simulink model "iot_casestudy_1_32"  (R2023a)
settings: Solver=VariableStepAuto  StartTime=0.0  StopTime=3.0  RelTol=1e-3
undefined symbols (not defined in the file or in its folder): m, n
(part 1 of 3)
settings Model: SimulationMode=accelerator  PacingRate=0.089000  Creator=simon  LastModifiedBy=simon
settings DataIOCC: SignalLogging=off
settings OptimizationCC: AccelVerboseBuild=on

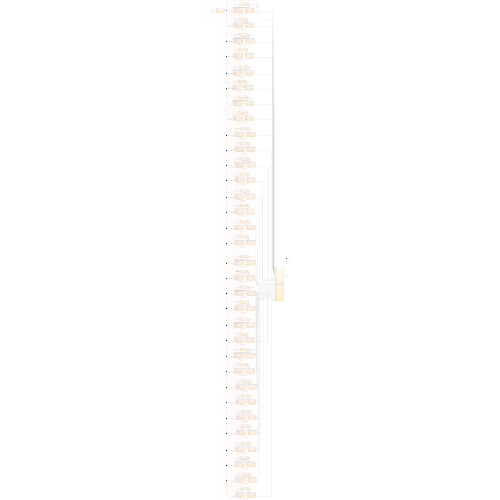
[thumbnail: Simulink's stored preview of the top-level diagram]
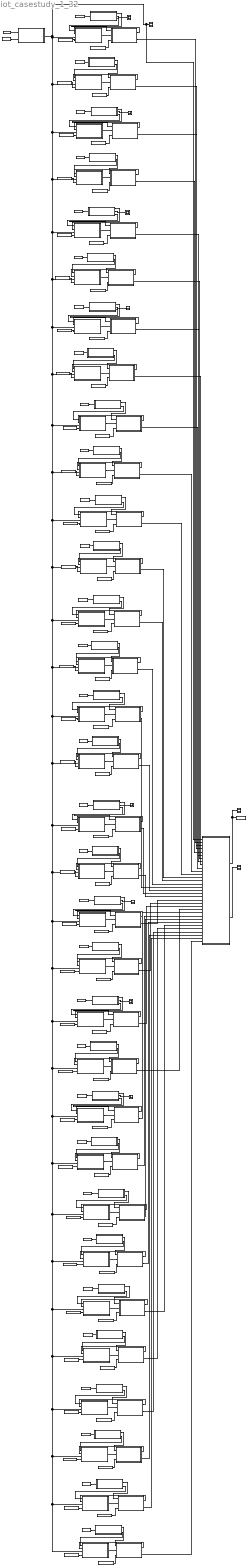
== system iot_casestudy_1_32 ==
  CameraControl : Stateflow chart  TreatAsAtomicUnit=on
      settings: PortSchema="{\"entries\":[{\"content\":{\"sides\":[{\"content\":{\"connectorIds\":[\"In3\",\"In1\",\"In2\"]},\"type\":\"ConnectorPlacement.EquallySpacedRectSide\",\"uuid\":\"ab620818-a51b-4a3c-9b00-600c4a6c30a0\"},{\"content\":{\"connectorIds\":[\"Out1\",\"Out2\"],\"side\":\"RIGHT\"},\"type\":\"ConnectorPlacement.EquallySpacedRectSide\",\"uuid\":\"fd7d4612-1aa1-44dc-acf4-0ffdcf3f06ab\"},{\"content\":{\"side\":\"TOP\"},\"type\":\"ConnectorPlacement.EquallySpacedRectSide\",\"uuid\":\"b173ad78-f658-4e97-9d6b-ed1d410de5f1\"}]},\"type\":\"ConnectorPlacement.EquallySpacedConnector\",\"uuid\":\"5700aeec-8725-4d1d-b13d-0f47828af58c\"}],\"packageUris\":[\"http://schema.mathworks.com/mf0/Connector/R2020b\"],\"version\":\"1.0\"}"
  CameraControl1 : Stateflow chart  TreatAsAtomicUnit=on
      settings: PortSchema="{\"entries\":[{\"content\":{\"sides\":[{\"content\":{\"connectorIds\":[\"In3\",\"In1\",\"In2\"]},\"type\":\"ConnectorPlacement.EquallySpacedRectSide\",\"uuid\":\"ab620818-a51b-4a3c-9b00-600c4a6c30a0\"},{\"content\":{\"connectorIds\":[\"Out1\",\"Out2\"],\"side\":\"RIGHT\"},\"type\":\"ConnectorPlacement.EquallySpacedRectSide\",\"uuid\":\"fd7d4612-1aa1-44dc-acf4-0ffdcf3f06ab\"},{\"content\":{\"side\":\"TOP\"},\"type\":\"ConnectorPlacement.EquallySpacedRectSide\",\"uuid\":\"b173ad78-f658-4e97-9d6b-ed1d410de5f1\"}]},\"type\":\"ConnectorPlacement.EquallySpacedConnector\",\"uuid\":\"5700aeec-8725-4d1d-b13d-0f47828af58c\"}],\"packageUris\":[\"http://schema.mathworks.com/mf0/Connector/R2020b\"],\"version\":\"1.0\"}"
  CameraControl10 : Stateflow chart  TreatAsAtomicUnit=on
      settings: PortSchema="{\"entries\":[{\"content\":{\"sides\":[{\"content\":{\"connectorIds\":[\"In3\",\"In1\",\"In2\"]},\"type\":\"ConnectorPlacement.EquallySpacedRectSide\",\"uuid\":\"ab620818-a51b-4a3c-9b00-600c4a6c30a0\"},{\"content\":{\"connectorIds\":[\"Out1\",\"Out2\"],\"side\":\"RIGHT\"},\"type\":\"ConnectorPlacement.EquallySpacedRectSide\",\"uuid\":\"fd7d4612-1aa1-44dc-acf4-0ffdcf3f06ab\"},{\"content\":{\"side\":\"TOP\"},\"type\":\"ConnectorPlacement.EquallySpacedRectSide\",\"uuid\":\"b173ad78-f658-4e97-9d6b-ed1d410de5f1\"}]},\"type\":\"ConnectorPlacement.EquallySpacedConnector\",\"uuid\":\"5700aeec-8725-4d1d-b13d-0f47828af58c\"}],\"packageUris\":[\"http://schema.mathworks.com/mf0/Connector/R2020b\"],\"version\":\"1.0\"}"
  CameraControl11 : Stateflow chart  TreatAsAtomicUnit=on
      settings: PortSchema="{\"entries\":[{\"content\":{\"sides\":[{\"content\":{\"connectorIds\":[\"In3\",\"In1\",\"In2\"]},\"type\":\"ConnectorPlacement.EquallySpacedRectSide\",\"uuid\":\"ab620818-a51b-4a3c-9b00-600c4a6c30a0\"},{\"content\":{\"connectorIds\":[\"Out1\",\"Out2\"],\"side\":\"RIGHT\"},\"type\":\"ConnectorPlacement.EquallySpacedRectSide\",\"uuid\":\"fd7d4612-1aa1-44dc-acf4-0ffdcf3f06ab\"},{\"content\":{\"side\":\"TOP\"},\"type\":\"ConnectorPlacement.EquallySpacedRectSide\",\"uuid\":\"b173ad78-f658-4e97-9d6b-ed1d410de5f1\"}]},\"type\":\"ConnectorPlacement.EquallySpacedConnector\",\"uuid\":\"5700aeec-8725-4d1d-b13d-0f47828af58c\"}],\"packageUris\":[\"http://schema.mathworks.com/mf0/Connector/R2020b\"],\"version\":\"1.0\"}"
  CameraControl12 : Stateflow chart  TreatAsAtomicUnit=on
      settings: PortSchema="{\"entries\":[{\"content\":{\"sides\":[{\"content\":{\"connectorIds\":[\"In3\",\"In1\",\"In2\"]},\"type\":\"ConnectorPlacement.EquallySpacedRectSide\",\"uuid\":\"ab620818-a51b-4a3c-9b00-600c4a6c30a0\"},{\"content\":{\"connectorIds\":[\"Out1\",\"Out2\"],\"side\":\"RIGHT\"},\"type\":\"ConnectorPlacement.EquallySpacedRectSide\",\"uuid\":\"fd7d4612-1aa1-44dc-acf4-0ffdcf3f06ab\"},{\"content\":{\"side\":\"TOP\"},\"type\":\"ConnectorPlacement.EquallySpacedRectSide\",\"uuid\":\"b173ad78-f658-4e97-9d6b-ed1d410de5f1\"}]},\"type\":\"ConnectorPlacement.EquallySpacedConnector\",\"uuid\":\"5700aeec-8725-4d1d-b13d-0f47828af58c\"}],\"packageUris\":[\"http://schema.mathworks.com/mf0/Connector/R2020b\"],\"version\":\"1.0\"}"
  CameraControl13 : Stateflow chart  TreatAsAtomicUnit=on
      settings: PortSchema="{\"entries\":[{\"content\":{\"sides\":[{\"content\":{\"connectorIds\":[\"In3\",\"In1\",\"In2\"]},\"type\":\"ConnectorPlacement.EquallySpacedRectSide\",\"uuid\":\"ab620818-a51b-4a3c-9b00-600c4a6c30a0\"},{\"content\":{\"connectorIds\":[\"Out1\",\"Out2\"],\"side\":\"RIGHT\"},\"type\":\"ConnectorPlacement.EquallySpacedRectSide\",\"uuid\":\"fd7d4612-1aa1-44dc-acf4-0ffdcf3f06ab\"},{\"content\":{\"side\":\"TOP\"},\"type\":\"ConnectorPlacement.EquallySpacedRectSide\",\"uuid\":\"b173ad78-f658-4e97-9d6b-ed1d410de5f1\"}]},\"type\":\"ConnectorPlacement.EquallySpacedConnector\",\"uuid\":\"5700aeec-8725-4d1d-b13d-0f47828af58c\"}],\"packageUris\":[\"http://schema.mathworks.com/mf0/Connector/R2020b\"],\"version\":\"1.0\"}"
  CameraControl14 : Stateflow chart  TreatAsAtomicUnit=on
      settings: PortSchema="{\"entries\":[{\"content\":{\"sides\":[{\"content\":{\"connectorIds\":[\"In3\",\"In1\",\"In2\"]},\"type\":\"ConnectorPlacement.EquallySpacedRectSide\",\"uuid\":\"ab620818-a51b-4a3c-9b00-600c4a6c30a0\"},{\"content\":{\"connectorIds\":[\"Out1\",\"Out2\"],\"side\":\"RIGHT\"},\"type\":\"ConnectorPlacement.EquallySpacedRectSide\",\"uuid\":\"fd7d4612-1aa1-44dc-acf4-0ffdcf3f06ab\"},{\"content\":{\"side\":\"TOP\"},\"type\":\"ConnectorPlacement.EquallySpacedRectSide\",\"uuid\":\"b173ad78-f658-4e97-9d6b-ed1d410de5f1\"}]},\"type\":\"ConnectorPlacement.EquallySpacedConnector\",\"uuid\":\"5700aeec-8725-4d1d-b13d-0f47828af58c\"}],\"packageUris\":[\"http://schema.mathworks.com/mf0/Connector/R2020b\"],\"version\":\"1.0\"}"
  CameraControl15 : Stateflow chart  TreatAsAtomicUnit=on
      settings: PortSchema="{\"entries\":[{\"content\":{\"sides\":[{\"content\":{\"connectorIds\":[\"In3\",\"In1\",\"In2\"]},\"type\":\"ConnectorPlacement.EquallySpacedRectSide\",\"uuid\":\"ab620818-a51b-4a3c-9b00-600c4a6c30a0\"},{\"content\":{\"connectorIds\":[\"Out1\",\"Out2\"],\"side\":\"RIGHT\"},\"type\":\"ConnectorPlacement.EquallySpacedRectSide\",\"uuid\":\"fd7d4612-1aa1-44dc-acf4-0ffdcf3f06ab\"},{\"content\":{\"side\":\"TOP\"},\"type\":\"ConnectorPlacement.EquallySpacedRectSide\",\"uuid\":\"b173ad78-f658-4e97-9d6b-ed1d410de5f1\"}]},\"type\":\"ConnectorPlacement.EquallySpacedConnector\",\"uuid\":\"5700aeec-8725-4d1d-b13d-0f47828af58c\"}],\"packageUris\":[\"http://schema.mathworks.com/mf0/Connector/R2020b\"],\"version\":\"1.0\"}"
  CameraControl16 : Stateflow chart  TreatAsAtomicUnit=on
      settings: PortSchema="{\"entries\":[{\"content\":{\"sides\":[{\"content\":{\"connectorIds\":[\"In3\",\"In1\",\"In2\"]},\"type\":\"ConnectorPlacement.EquallySpacedRectSide\",\"uuid\":\"ab620818-a51b-4a3c-9b00-600c4a6c30a0\"},{\"content\":{\"connectorIds\":[\"Out1\",\"Out2\"],\"side\":\"RIGHT\"},\"type\":\"ConnectorPlacement.EquallySpacedRectSide\",\"uuid\":\"fd7d4612-1aa1-44dc-acf4-0ffdcf3f06ab\"},{\"content\":{\"side\":\"TOP\"},\"type\":\"ConnectorPlacement.EquallySpacedRectSide\",\"uuid\":\"b173ad78-f658-4e97-9d6b-ed1d410de5f1\"}]},\"type\":\"ConnectorPlacement.EquallySpacedConnector\",\"uuid\":\"5700aeec-8725-4d1d-b13d-0f47828af58c\"}],\"packageUris\":[\"http://schema.mathworks.com/mf0/Connector/R2020b\"],\"version\":\"1.0\"}"
  CameraControl17 : Stateflow chart  TreatAsAtomicUnit=on
      settings: PortSchema="{\"entries\":[{\"content\":{\"sides\":[{\"content\":{\"connectorIds\":[\"In3\",\"In1\",\"In2\"]},\"type\":\"ConnectorPlacement.EquallySpacedRectSide\",\"uuid\":\"ab620818-a51b-4a3c-9b00-600c4a6c30a0\"},{\"content\":{\"connectorIds\":[\"Out1\",\"Out2\"],\"side\":\"RIGHT\"},\"type\":\"ConnectorPlacement.EquallySpacedRectSide\",\"uuid\":\"fd7d4612-1aa1-44dc-acf4-0ffdcf3f06ab\"},{\"content\":{\"side\":\"TOP\"},\"type\":\"ConnectorPlacement.EquallySpacedRectSide\",\"uuid\":\"b173ad78-f658-4e97-9d6b-ed1d410de5f1\"}]},\"type\":\"ConnectorPlacement.EquallySpacedConnector\",\"uuid\":\"5700aeec-8725-4d1d-b13d-0f47828af58c\"}],\"packageUris\":[\"http://schema.mathworks.com/mf0/Connector/R2020b\"],\"version\":\"1.0\"}"
  CameraControl18 : Stateflow chart  TreatAsAtomicUnit=on
      settings: PortSchema="{\"entries\":[{\"content\":{\"sides\":[{\"content\":{\"connectorIds\":[\"In3\",\"In1\",\"In2\"]},\"type\":\"ConnectorPlacement.EquallySpacedRectSide\",\"uuid\":\"ab620818-a51b-4a3c-9b00-600c4a6c30a0\"},{\"content\":{\"connectorIds\":[\"Out1\",\"Out2\"],\"side\":\"RIGHT\"},\"type\":\"ConnectorPlacement.EquallySpacedRectSide\",\"uuid\":\"fd7d4612-1aa1-44dc-acf4-0ffdcf3f06ab\"},{\"content\":{\"side\":\"TOP\"},\"type\":\"ConnectorPlacement.EquallySpacedRectSide\",\"uuid\":\"b173ad78-f658-4e97-9d6b-ed1d410de5f1\"}]},\"type\":\"ConnectorPlacement.EquallySpacedConnector\",\"uuid\":\"5700aeec-8725-4d1d-b13d-0f47828af58c\"}],\"packageUris\":[\"http://schema.mathworks.com/mf0/Connector/R2020b\"],\"version\":\"1.0\"}"
  CameraControl19 : Stateflow chart  TreatAsAtomicUnit=on
      settings: PortSchema="{\"entries\":[{\"content\":{\"sides\":[{\"content\":{\"connectorIds\":[\"In3\",\"In1\",\"In2\"]},\"type\":\"ConnectorPlacement.EquallySpacedRectSide\",\"uuid\":\"ab620818-a51b-4a3c-9b00-600c4a6c30a0\"},{\"content\":{\"connectorIds\":[\"Out1\",\"Out2\"],\"side\":\"RIGHT\"},\"type\":\"ConnectorPlacement.EquallySpacedRectSide\",\"uuid\":\"fd7d4612-1aa1-44dc-acf4-0ffdcf3f06ab\"},{\"content\":{\"side\":\"TOP\"},\"type\":\"ConnectorPlacement.EquallySpacedRectSide\",\"uuid\":\"b173ad78-f658-4e97-9d6b-ed1d410de5f1\"}]},\"type\":\"ConnectorPlacement.EquallySpacedConnector\",\"uuid\":\"5700aeec-8725-4d1d-b13d-0f47828af58c\"}],\"packageUris\":[\"http://schema.mathworks.com/mf0/Connector/R2020b\"],\"version\":\"1.0\"}"
  CameraControl2 : Stateflow chart  TreatAsAtomicUnit=on
      settings: PortSchema="{\"entries\":[{\"content\":{\"sides\":[{\"content\":{\"connectorIds\":[\"In3\",\"In1\",\"In2\"]},\"type\":\"ConnectorPlacement.EquallySpacedRectSide\",\"uuid\":\"ab620818-a51b-4a3c-9b00-600c4a6c30a0\"},{\"content\":{\"connectorIds\":[\"Out1\",\"Out2\"],\"side\":\"RIGHT\"},\"type\":\"ConnectorPlacement.EquallySpacedRectSide\",\"uuid\":\"fd7d4612-1aa1-44dc-acf4-0ffdcf3f06ab\"},{\"content\":{\"side\":\"TOP\"},\"type\":\"ConnectorPlacement.EquallySpacedRectSide\",\"uuid\":\"b173ad78-f658-4e97-9d6b-ed1d410de5f1\"}]},\"type\":\"ConnectorPlacement.EquallySpacedConnector\",\"uuid\":\"5700aeec-8725-4d1d-b13d-0f47828af58c\"}],\"packageUris\":[\"http://schema.mathworks.com/mf0/Connector/R2020b\"],\"version\":\"1.0\"}"
  CameraControl20 : Stateflow chart  TreatAsAtomicUnit=on
      settings: PortSchema="{\"entries\":[{\"content\":{\"sides\":[{\"content\":{\"connectorIds\":[\"In3\",\"In1\",\"In2\"]},\"type\":\"ConnectorPlacement.EquallySpacedRectSide\",\"uuid\":\"ab620818-a51b-4a3c-9b00-600c4a6c30a0\"},{\"content\":{\"connectorIds\":[\"Out1\",\"Out2\"],\"side\":\"RIGHT\"},\"type\":\"ConnectorPlacement.EquallySpacedRectSide\",\"uuid\":\"fd7d4612-1aa1-44dc-acf4-0ffdcf3f06ab\"},{\"content\":{\"side\":\"TOP\"},\"type\":\"ConnectorPlacement.EquallySpacedRectSide\",\"uuid\":\"b173ad78-f658-4e97-9d6b-ed1d410de5f1\"}]},\"type\":\"ConnectorPlacement.EquallySpacedConnector\",\"uuid\":\"5700aeec-8725-4d1d-b13d-0f47828af58c\"}],\"packageUris\":[\"http://schema.mathworks.com/mf0/Connector/R2020b\"],\"version\":\"1.0\"}"
  CameraControl21 : Stateflow chart  TreatAsAtomicUnit=on
      settings: PortSchema="{\"entries\":[{\"content\":{\"sides\":[{\"content\":{\"connectorIds\":[\"In3\",\"In1\",\"In2\"]},\"type\":\"ConnectorPlacement.EquallySpacedRectSide\",\"uuid\":\"ab620818-a51b-4a3c-9b00-600c4a6c30a0\"},{\"content\":{\"connectorIds\":[\"Out1\",\"Out2\"],\"side\":\"RIGHT\"},\"type\":\"ConnectorPlacement.EquallySpacedRectSide\",\"uuid\":\"fd7d4612-1aa1-44dc-acf4-0ffdcf3f06ab\"},{\"content\":{\"side\":\"TOP\"},\"type\":\"ConnectorPlacement.EquallySpacedRectSide\",\"uuid\":\"b173ad78-f658-4e97-9d6b-ed1d410de5f1\"}]},\"type\":\"ConnectorPlacement.EquallySpacedConnector\",\"uuid\":\"5700aeec-8725-4d1d-b13d-0f47828af58c\"}],\"packageUris\":[\"http://schema.mathworks.com/mf0/Connector/R2020b\"],\"version\":\"1.0\"}"
  CameraControl22 : Stateflow chart  TreatAsAtomicUnit=on
      settings: PortSchema="{\"entries\":[{\"content\":{\"sides\":[{\"content\":{\"connectorIds\":[\"In3\",\"In1\",\"In2\"]},\"type\":\"ConnectorPlacement.EquallySpacedRectSide\",\"uuid\":\"ab620818-a51b-4a3c-9b00-600c4a6c30a0\"},{\"content\":{\"connectorIds\":[\"Out1\",\"Out2\"],\"side\":\"RIGHT\"},\"type\":\"ConnectorPlacement.EquallySpacedRectSide\",\"uuid\":\"fd7d4612-1aa1-44dc-acf4-0ffdcf3f06ab\"},{\"content\":{\"side\":\"TOP\"},\"type\":\"ConnectorPlacement.EquallySpacedRectSide\",\"uuid\":\"b173ad78-f658-4e97-9d6b-ed1d410de5f1\"}]},\"type\":\"ConnectorPlacement.EquallySpacedConnector\",\"uuid\":\"5700aeec-8725-4d1d-b13d-0f47828af58c\"}],\"packageUris\":[\"http://schema.mathworks.com/mf0/Connector/R2020b\"],\"version\":\"1.0\"}"
  CameraControl23 : Stateflow chart  TreatAsAtomicUnit=on
      settings: PortSchema="{\"entries\":[{\"content\":{\"sides\":[{\"content\":{\"connectorIds\":[\"In3\",\"In1\",\"In2\"]},\"type\":\"ConnectorPlacement.EquallySpacedRectSide\",\"uuid\":\"ab620818-a51b-4a3c-9b00-600c4a6c30a0\"},{\"content\":{\"connectorIds\":[\"Out1\",\"Out2\"],\"side\":\"RIGHT\"},\"type\":\"ConnectorPlacement.EquallySpacedRectSide\",\"uuid\":\"fd7d4612-1aa1-44dc-acf4-0ffdcf3f06ab\"},{\"content\":{\"side\":\"TOP\"},\"type\":\"ConnectorPlacement.EquallySpacedRectSide\",\"uuid\":\"b173ad78-f658-4e97-9d6b-ed1d410de5f1\"}]},\"type\":\"ConnectorPlacement.EquallySpacedConnector\",\"uuid\":\"5700aeec-8725-4d1d-b13d-0f47828af58c\"}],\"packageUris\":[\"http://schema.mathworks.com/mf0/Connector/R2020b\"],\"version\":\"1.0\"}"
  CameraControl24 : Stateflow chart  TreatAsAtomicUnit=on
      settings: PortSchema="{\"entries\":[{\"content\":{\"sides\":[{\"content\":{\"connectorIds\":[\"In3\",\"In1\",\"In2\"]},\"type\":\"ConnectorPlacement.EquallySpacedRectSide\",\"uuid\":\"ab620818-a51b-4a3c-9b00-600c4a6c30a0\"},{\"content\":{\"connectorIds\":[\"Out1\",\"Out2\"],\"side\":\"RIGHT\"},\"type\":\"ConnectorPlacement.EquallySpacedRectSide\",\"uuid\":\"fd7d4612-1aa1-44dc-acf4-0ffdcf3f06ab\"},{\"content\":{\"side\":\"TOP\"},\"type\":\"ConnectorPlacement.EquallySpacedRectSide\",\"uuid\":\"b173ad78-f658-4e97-9d6b-ed1d410de5f1\"}]},\"type\":\"ConnectorPlacement.EquallySpacedConnector\",\"uuid\":\"5700aeec-8725-4d1d-b13d-0f47828af58c\"}],\"packageUris\":[\"http://schema.mathworks.com/mf0/Connector/R2020b\"],\"version\":\"1.0\"}"
  CameraControl25 : Stateflow chart  TreatAsAtomicUnit=on
      settings: PortSchema="{\"entries\":[{\"content\":{\"sides\":[{\"content\":{\"connectorIds\":[\"In3\",\"In1\",\"In2\"]},\"type\":\"ConnectorPlacement.EquallySpacedRectSide\",\"uuid\":\"ab620818-a51b-4a3c-9b00-600c4a6c30a0\"},{\"content\":{\"connectorIds\":[\"Out1\",\"Out2\"],\"side\":\"RIGHT\"},\"type\":\"ConnectorPlacement.EquallySpacedRectSide\",\"uuid\":\"fd7d4612-1aa1-44dc-acf4-0ffdcf3f06ab\"},{\"content\":{\"side\":\"TOP\"},\"type\":\"ConnectorPlacement.EquallySpacedRectSide\",\"uuid\":\"b173ad78-f658-4e97-9d6b-ed1d410de5f1\"}]},\"type\":\"ConnectorPlacement.EquallySpacedConnector\",\"uuid\":\"5700aeec-8725-4d1d-b13d-0f47828af58c\"}],\"packageUris\":[\"http://schema.mathworks.com/mf0/Connector/R2020b\"],\"version\":\"1.0\"}"
  CameraControl26 : Stateflow chart  TreatAsAtomicUnit=on
      settings: PortSchema="{\"entries\":[{\"content\":{\"sides\":[{\"content\":{\"connectorIds\":[\"In3\",\"In1\",\"In2\"]},\"type\":\"ConnectorPlacement.EquallySpacedRectSide\",\"uuid\":\"ab620818-a51b-4a3c-9b00-600c4a6c30a0\"},{\"content\":{\"connectorIds\":[\"Out1\",\"Out2\"],\"side\":\"RIGHT\"},\"type\":\"ConnectorPlacement.EquallySpacedRectSide\",\"uuid\":\"fd7d4612-1aa1-44dc-acf4-0ffdcf3f06ab\"},{\"content\":{\"side\":\"TOP\"},\"type\":\"ConnectorPlacement.EquallySpacedRectSide\",\"uuid\":\"b173ad78-f658-4e97-9d6b-ed1d410de5f1\"}]},\"type\":\"ConnectorPlacement.EquallySpacedConnector\",\"uuid\":\"5700aeec-8725-4d1d-b13d-0f47828af58c\"}],\"packageUris\":[\"http://schema.mathworks.com/mf0/Connector/R2020b\"],\"version\":\"1.0\"}"
  CameraControl27 : Stateflow chart  TreatAsAtomicUnit=on
      settings: PortSchema="{\"entries\":[{\"content\":{\"sides\":[{\"content\":{\"connectorIds\":[\"In3\",\"In1\",\"In2\"]},\"type\":\"ConnectorPlacement.EquallySpacedRectSide\",\"uuid\":\"ab620818-a51b-4a3c-9b00-600c4a6c30a0\"},{\"content\":{\"connectorIds\":[\"Out1\",\"Out2\"],\"side\":\"RIGHT\"},\"type\":\"ConnectorPlacement.EquallySpacedRectSide\",\"uuid\":\"fd7d4612-1aa1-44dc-acf4-0ffdcf3f06ab\"},{\"content\":{\"side\":\"TOP\"},\"type\":\"ConnectorPlacement.EquallySpacedRectSide\",\"uuid\":\"b173ad78-f658-4e97-9d6b-ed1d410de5f1\"}]},\"type\":\"ConnectorPlacement.EquallySpacedConnector\",\"uuid\":\"5700aeec-8725-4d1d-b13d-0f47828af58c\"}],\"packageUris\":[\"http://schema.mathworks.com/mf0/Connector/R2020b\"],\"version\":\"1.0\"}"
  CameraControl28 : Stateflow chart  TreatAsAtomicUnit=on
      settings: PortSchema="{\"entries\":[{\"content\":{\"sides\":[{\"content\":{\"connectorIds\":[\"In3\",\"In1\",\"In2\"]},\"type\":\"ConnectorPlacement.EquallySpacedRectSide\",\"uuid\":\"ab620818-a51b-4a3c-9b00-600c4a6c30a0\"},{\"content\":{\"connectorIds\":[\"Out1\",\"Out2\"],\"side\":\"RIGHT\"},\"type\":\"ConnectorPlacement.EquallySpacedRectSide\",\"uuid\":\"fd7d4612-1aa1-44dc-acf4-0ffdcf3f06ab\"},{\"content\":{\"side\":\"TOP\"},\"type\":\"ConnectorPlacement.EquallySpacedRectSide\",\"uuid\":\"b173ad78-f658-4e97-9d6b-ed1d410de5f1\"}]},\"type\":\"ConnectorPlacement.EquallySpacedConnector\",\"uuid\":\"5700aeec-8725-4d1d-b13d-0f47828af58c\"}],\"packageUris\":[\"http://schema.mathworks.com/mf0/Connector/R2020b\"],\"version\":\"1.0\"}"
  CameraControl29 : Stateflow chart  TreatAsAtomicUnit=on
      settings: PortSchema="{\"entries\":[{\"content\":{\"sides\":[{\"content\":{\"connectorIds\":[\"In3\",\"In1\",\"In2\"]},\"type\":\"ConnectorPlacement.EquallySpacedRectSide\",\"uuid\":\"ab620818-a51b-4a3c-9b00-600c4a6c30a0\"},{\"content\":{\"connectorIds\":[\"Out1\",\"Out2\"],\"side\":\"RIGHT\"},\"type\":\"ConnectorPlacement.EquallySpacedRectSide\",\"uuid\":\"fd7d4612-1aa1-44dc-acf4-0ffdcf3f06ab\"},{\"content\":{\"side\":\"TOP\"},\"type\":\"ConnectorPlacement.EquallySpacedRectSide\",\"uuid\":\"b173ad78-f658-4e97-9d6b-ed1d410de5f1\"}]},\"type\":\"ConnectorPlacement.EquallySpacedConnector\",\"uuid\":\"5700aeec-8725-4d1d-b13d-0f47828af58c\"}],\"packageUris\":[\"http://schema.mathworks.com/mf0/Connector/R2020b\"],\"version\":\"1.0\"}"
  CameraControl3 : Stateflow chart  TreatAsAtomicUnit=on
      settings: PortSchema="{\"entries\":[{\"content\":{\"sides\":[{\"content\":{\"connectorIds\":[\"In3\",\"In1\",\"In2\"]},\"type\":\"ConnectorPlacement.EquallySpacedRectSide\",\"uuid\":\"ab620818-a51b-4a3c-9b00-600c4a6c30a0\"},{\"content\":{\"connectorIds\":[\"Out1\",\"Out2\"],\"side\":\"RIGHT\"},\"type\":\"ConnectorPlacement.EquallySpacedRectSide\",\"uuid\":\"fd7d4612-1aa1-44dc-acf4-0ffdcf3f06ab\"},{\"content\":{\"side\":\"TOP\"},\"type\":\"ConnectorPlacement.EquallySpacedRectSide\",\"uuid\":\"b173ad78-f658-4e97-9d6b-ed1d410de5f1\"}]},\"type\":\"ConnectorPlacement.EquallySpacedConnector\",\"uuid\":\"5700aeec-8725-4d1d-b13d-0f47828af58c\"}],\"packageUris\":[\"http://schema.mathworks.com/mf0/Connector/R2020b\"],\"version\":\"1.0\"}"
  CameraControl30 : Stateflow chart  TreatAsAtomicUnit=on
      settings: PortSchema="{\"entries\":[{\"content\":{\"sides\":[{\"content\":{\"connectorIds\":[\"In3\",\"In1\",\"In2\"]},\"type\":\"ConnectorPlacement.EquallySpacedRectSide\",\"uuid\":\"ab620818-a51b-4a3c-9b00-600c4a6c30a0\"},{\"content\":{\"connectorIds\":[\"Out1\",\"Out2\"],\"side\":\"RIGHT\"},\"type\":\"ConnectorPlacement.EquallySpacedRectSide\",\"uuid\":\"fd7d4612-1aa1-44dc-acf4-0ffdcf3f06ab\"},{\"content\":{\"side\":\"TOP\"},\"type\":\"ConnectorPlacement.EquallySpacedRectSide\",\"uuid\":\"b173ad78-f658-4e97-9d6b-ed1d410de5f1\"}]},\"type\":\"ConnectorPlacement.EquallySpacedConnector\",\"uuid\":\"5700aeec-8725-4d1d-b13d-0f47828af58c\"}],\"packageUris\":[\"http://schema.mathworks.com/mf0/Connector/R2020b\"],\"version\":\"1.0\"}"
  CameraControl31 : Stateflow chart  TreatAsAtomicUnit=on
      settings: PortSchema="{\"entries\":[{\"content\":{\"sides\":[{\"content\":{\"connectorIds\":[\"In3\",\"In1\",\"In2\"]},\"type\":\"ConnectorPlacement.EquallySpacedRectSide\",\"uuid\":\"ab620818-a51b-4a3c-9b00-600c4a6c30a0\"},{\"content\":{\"connectorIds\":[\"Out1\",\"Out2\"],\"side\":\"RIGHT\"},\"type\":\"ConnectorPlacement.EquallySpacedRectSide\",\"uuid\":\"fd7d4612-1aa1-44dc-acf4-0ffdcf3f06ab\"},{\"content\":{\"side\":\"TOP\"},\"type\":\"ConnectorPlacement.EquallySpacedRectSide\",\"uuid\":\"b173ad78-f658-4e97-9d6b-ed1d410de5f1\"}]},\"type\":\"ConnectorPlacement.EquallySpacedConnector\",\"uuid\":\"5700aeec-8725-4d1d-b13d-0f47828af58c\"}],\"packageUris\":[\"http://schema.mathworks.com/mf0/Connector/R2020b\"],\"version\":\"1.0\"}"
  CameraControl4 : Stateflow chart  TreatAsAtomicUnit=on
      settings: PortSchema="{\"entries\":[{\"content\":{\"sides\":[{\"content\":{\"connectorIds\":[\"In3\",\"In1\",\"In2\"]},\"type\":\"ConnectorPlacement.EquallySpacedRectSide\",\"uuid\":\"ab620818-a51b-4a3c-9b00-600c4a6c30a0\"},{\"content\":{\"connectorIds\":[\"Out1\",\"Out2\"],\"side\":\"RIGHT\"},\"type\":\"ConnectorPlacement.EquallySpacedRectSide\",\"uuid\":\"fd7d4612-1aa1-44dc-acf4-0ffdcf3f06ab\"},{\"content\":{\"side\":\"TOP\"},\"type\":\"ConnectorPlacement.EquallySpacedRectSide\",\"uuid\":\"b173ad78-f658-4e97-9d6b-ed1d410de5f1\"}]},\"type\":\"ConnectorPlacement.EquallySpacedConnector\",\"uuid\":\"5700aeec-8725-4d1d-b13d-0f47828af58c\"}],\"packageUris\":[\"http://schema.mathworks.com/mf0/Connector/R2020b\"],\"version\":\"1.0\"}"
  CameraControl5 : Stateflow chart  TreatAsAtomicUnit=on
      settings: PortSchema="{\"entries\":[{\"content\":{\"sides\":[{\"content\":{\"connectorIds\":[\"In3\",\"In1\",\"In2\"]},\"type\":\"ConnectorPlacement.EquallySpacedRectSide\",\"uuid\":\"ab620818-a51b-4a3c-9b00-600c4a6c30a0\"},{\"content\":{\"connectorIds\":[\"Out1\",\"Out2\"],\"side\":\"RIGHT\"},\"type\":\"ConnectorPlacement.EquallySpacedRectSide\",\"uuid\":\"fd7d4612-1aa1-44dc-acf4-0ffdcf3f06ab\"},{\"content\":{\"side\":\"TOP\"},\"type\":\"ConnectorPlacement.EquallySpacedRectSide\",\"uuid\":\"b173ad78-f658-4e97-9d6b-ed1d410de5f1\"}]},\"type\":\"ConnectorPlacement.EquallySpacedConnector\",\"uuid\":\"5700aeec-8725-4d1d-b13d-0f47828af58c\"}],\"packageUris\":[\"http://schema.mathworks.com/mf0/Connector/R2020b\"],\"version\":\"1.0\"}"
  CameraControl6 : Stateflow chart  TreatAsAtomicUnit=on
      settings: PortSchema="{\"entries\":[{\"content\":{\"sides\":[{\"content\":{\"connectorIds\":[\"In3\",\"In1\",\"In2\"]},\"type\":\"ConnectorPlacement.EquallySpacedRectSide\",\"uuid\":\"ab620818-a51b-4a3c-9b00-600c4a6c30a0\"},{\"content\":{\"connectorIds\":[\"Out1\",\"Out2\"],\"side\":\"RIGHT\"},\"type\":\"ConnectorPlacement.EquallySpacedRectSide\",\"uuid\":\"fd7d4612-1aa1-44dc-acf4-0ffdcf3f06ab\"},{\"content\":{\"side\":\"TOP\"},\"type\":\"ConnectorPlacement.EquallySpacedRectSide\",\"uuid\":\"b173ad78-f658-4e97-9d6b-ed1d410de5f1\"}]},\"type\":\"ConnectorPlacement.EquallySpacedConnector\",\"uuid\":\"5700aeec-8725-4d1d-b13d-0f47828af58c\"}],\"packageUris\":[\"http://schema.mathworks.com/mf0/Connector/R2020b\"],\"version\":\"1.0\"}"
  CameraControl7 : Stateflow chart  TreatAsAtomicUnit=on
      settings: PortSchema="{\"entries\":[{\"content\":{\"sides\":[{\"content\":{\"connectorIds\":[\"In3\",\"In1\",\"In2\"]},\"type\":\"ConnectorPlacement.EquallySpacedRectSide\",\"uuid\":\"ab620818-a51b-4a3c-9b00-600c4a6c30a0\"},{\"content\":{\"connectorIds\":[\"Out1\",\"Out2\"],\"side\":\"RIGHT\"},\"type\":\"ConnectorPlacement.EquallySpacedRectSide\",\"uuid\":\"fd7d4612-1aa1-44dc-acf4-0ffdcf3f06ab\"},{\"content\":{\"side\":\"TOP\"},\"type\":\"ConnectorPlacement.EquallySpacedRectSide\",\"uuid\":\"b173ad78-f658-4e97-9d6b-ed1d410de5f1\"}]},\"type\":\"ConnectorPlacement.EquallySpacedConnector\",\"uuid\":\"5700aeec-8725-4d1d-b13d-0f47828af58c\"}],\"packageUris\":[\"http://schema.mathworks.com/mf0/Connector/R2020b\"],\"version\":\"1.0\"}"
  CameraControl8 : Stateflow chart  TreatAsAtomicUnit=on
      settings: PortSchema="{\"entries\":[{\"content\":{\"sides\":[{\"content\":{\"connectorIds\":[\"In3\",\"In1\",\"In2\"]},\"type\":\"ConnectorPlacement.EquallySpacedRectSide\",\"uuid\":\"ab620818-a51b-4a3c-9b00-600c4a6c30a0\"},{\"content\":{\"connectorIds\":[\"Out1\",\"Out2\"],\"side\":\"RIGHT\"},\"type\":\"ConnectorPlacement.EquallySpacedRectSide\",\"uuid\":\"fd7d4612-1aa1-44dc-acf4-0ffdcf3f06ab\"},{\"content\":{\"side\":\"TOP\"},\"type\":\"ConnectorPlacement.EquallySpacedRectSide\",\"uuid\":\"b173ad78-f658-4e97-9d6b-ed1d410de5f1\"}]},\"type\":\"ConnectorPlacement.EquallySpacedConnector\",\"uuid\":\"5700aeec-8725-4d1d-b13d-0f47828af58c\"}],\"packageUris\":[\"http://schema.mathworks.com/mf0/Connector/R2020b\"],\"version\":\"1.0\"}"
  CameraControl9 : Stateflow chart  TreatAsAtomicUnit=on
      settings: PortSchema="{\"entries\":[{\"content\":{\"sides\":[{\"content\":{\"connectorIds\":[\"In3\",\"In1\",\"In2\"]},\"type\":\"ConnectorPlacement.EquallySpacedRectSide\",\"uuid\":\"ab620818-a51b-4a3c-9b00-600c4a6c30a0\"},{\"content\":{\"connectorIds\":[\"Out1\",\"Out2\"],\"side\":\"RIGHT\"},\"type\":\"ConnectorPlacement.EquallySpacedRectSide\",\"uuid\":\"fd7d4612-1aa1-44dc-acf4-0ffdcf3f06ab\"},{\"content\":{\"side\":\"TOP\"},\"type\":\"ConnectorPlacement.EquallySpacedRectSide\",\"uuid\":\"b173ad78-f658-4e97-9d6b-ed1d410de5f1\"}]},\"type\":\"ConnectorPlacement.EquallySpacedConnector\",\"uuid\":\"5700aeec-8725-4d1d-b13d-0f47828af58c\"}],\"packageUris\":[\"http://schema.mathworks.com/mf0/Connector/R2020b\"],\"version\":\"1.0\"}"
  CameraDriver : Stateflow chart  TreatAsAtomicUnit=on
      settings: PortSchema="{\"entries\":[{\"content\":{\"sides\":[{\"content\":{\"connectorIds\":[\"In4\",\"In1\",\"In2\",\"In3\"]},\"type\":\"ConnectorPlacement.EquallySpacedRectSide\",\"uuid\":\"49bdffc0-8e15-4462-b991-b36534669558\"},{\"content\":{\"connectorIds\":[\"Out1\"],\"side\":\"RIGHT\"},\"type\":\"ConnectorPlacement.EquallySpacedRectSide\",\"uuid\":\"379950e5-a8e3-41fb-8f45-c3d731cfbd8a\"},{\"content\":{\"side\":\"TOP\"},\"type\":\"ConnectorPlacement.EquallySpacedRectSide\",\"uuid\":\"38309075-1b62-4fbc-9171-ddac584f70df\"}]},\"type\":\"ConnectorPlacement.EquallySpacedConnector\",\"uuid\":\"335a78c7-f6bb-4aff-a350-269f860e2554\"}],\"packageUris\":[\"http://schema.mathworks.com/mf0/Connector/R2020b\"],\"version\":\"1.0\"}"
  CameraDriver1 : Stateflow chart  TreatAsAtomicUnit=on
      settings: PortSchema="{\"entries\":[{\"content\":{\"sides\":[{\"content\":{\"connectorIds\":[\"In4\",\"In1\",\"In2\",\"In3\"]},\"type\":\"ConnectorPlacement.EquallySpacedRectSide\",\"uuid\":\"49bdffc0-8e15-4462-b991-b36534669558\"},{\"content\":{\"connectorIds\":[\"Out1\"],\"side\":\"RIGHT\"},\"type\":\"ConnectorPlacement.EquallySpacedRectSide\",\"uuid\":\"379950e5-a8e3-41fb-8f45-c3d731cfbd8a\"},{\"content\":{\"side\":\"TOP\"},\"type\":\"ConnectorPlacement.EquallySpacedRectSide\",\"uuid\":\"38309075-1b62-4fbc-9171-ddac584f70df\"}]},\"type\":\"ConnectorPlacement.EquallySpacedConnector\",\"uuid\":\"335a78c7-f6bb-4aff-a350-269f860e2554\"}],\"packageUris\":[\"http://schema.mathworks.com/mf0/Connector/R2020b\"],\"version\":\"1.0\"}"
  CameraDriver10 : Stateflow chart  TreatAsAtomicUnit=on
      settings: PortSchema="{\"entries\":[{\"content\":{\"sides\":[{\"content\":{\"connectorIds\":[\"In4\",\"In1\",\"In2\",\"In3\"]},\"type\":\"ConnectorPlacement.EquallySpacedRectSide\",\"uuid\":\"49bdffc0-8e15-4462-b991-b36534669558\"},{\"content\":{\"connectorIds\":[\"Out1\"],\"side\":\"RIGHT\"},\"type\":\"ConnectorPlacement.EquallySpacedRectSide\",\"uuid\":\"379950e5-a8e3-41fb-8f45-c3d731cfbd8a\"},{\"content\":{\"side\":\"TOP\"},\"type\":\"ConnectorPlacement.EquallySpacedRectSide\",\"uuid\":\"38309075-1b62-4fbc-9171-ddac584f70df\"}]},\"type\":\"ConnectorPlacement.EquallySpacedConnector\",\"uuid\":\"335a78c7-f6bb-4aff-a350-269f860e2554\"}],\"packageUris\":[\"http://schema.mathworks.com/mf0/Connector/R2020b\"],\"version\":\"1.0\"}"
  CameraDriver11 : Stateflow chart  TreatAsAtomicUnit=on
      settings: PortSchema="{\"entries\":[{\"content\":{\"sides\":[{\"content\":{\"connectorIds\":[\"In4\",\"In1\",\"In2\",\"In3\"]},\"type\":\"ConnectorPlacement.EquallySpacedRectSide\",\"uuid\":\"49bdffc0-8e15-4462-b991-b36534669558\"},{\"content\":{\"connectorIds\":[\"Out1\"],\"side\":\"RIGHT\"},\"type\":\"ConnectorPlacement.EquallySpacedRectSide\",\"uuid\":\"379950e5-a8e3-41fb-8f45-c3d731cfbd8a\"},{\"content\":{\"side\":\"TOP\"},\"type\":\"ConnectorPlacement.EquallySpacedRectSide\",\"uuid\":\"38309075-1b62-4fbc-9171-ddac584f70df\"}]},\"type\":\"ConnectorPlacement.EquallySpacedConnector\",\"uuid\":\"335a78c7-f6bb-4aff-a350-269f860e2554\"}],\"packageUris\":[\"http://schema.mathworks.com/mf0/Connector/R2020b\"],\"version\":\"1.0\"}"
  CameraDriver12 : Stateflow chart  TreatAsAtomicUnit=on
      settings: PortSchema="{\"entries\":[{\"content\":{\"sides\":[{\"content\":{\"connectorIds\":[\"In4\",\"In1\",\"In2\",\"In3\"]},\"type\":\"ConnectorPlacement.EquallySpacedRectSide\",\"uuid\":\"49bdffc0-8e15-4462-b991-b36534669558\"},{\"content\":{\"connectorIds\":[\"Out1\"],\"side\":\"RIGHT\"},\"type\":\"ConnectorPlacement.EquallySpacedRectSide\",\"uuid\":\"379950e5-a8e3-41fb-8f45-c3d731cfbd8a\"},{\"content\":{\"side\":\"TOP\"},\"type\":\"ConnectorPlacement.EquallySpacedRectSide\",\"uuid\":\"38309075-1b62-4fbc-9171-ddac584f70df\"}]},\"type\":\"ConnectorPlacement.EquallySpacedConnector\",\"uuid\":\"335a78c7-f6bb-4aff-a350-269f860e2554\"}],\"packageUris\":[\"http://schema.mathworks.com/mf0/Connector/R2020b\"],\"version\":\"1.0\"}"
  CameraDriver13 : Stateflow chart  TreatAsAtomicUnit=on
      settings: PortSchema="{\"entries\":[{\"content\":{\"sides\":[{\"content\":{\"connectorIds\":[\"In4\",\"In1\",\"In2\",\"In3\"]},\"type\":\"ConnectorPlacement.EquallySpacedRectSide\",\"uuid\":\"49bdffc0-8e15-4462-b991-b36534669558\"},{\"content\":{\"connectorIds\":[\"Out1\"],\"side\":\"RIGHT\"},\"type\":\"ConnectorPlacement.EquallySpacedRectSide\",\"uuid\":\"379950e5-a8e3-41fb-8f45-c3d731cfbd8a\"},{\"content\":{\"side\":\"TOP\"},\"type\":\"ConnectorPlacement.EquallySpacedRectSide\",\"uuid\":\"38309075-1b62-4fbc-9171-ddac584f70df\"}]},\"type\":\"ConnectorPlacement.EquallySpacedConnector\",\"uuid\":\"335a78c7-f6bb-4aff-a350-269f860e2554\"}],\"packageUris\":[\"http://schema.mathworks.com/mf0/Connector/R2020b\"],\"version\":\"1.0\"}"
  CameraDriver14 : Stateflow chart  TreatAsAtomicUnit=on
      settings: PortSchema="{\"entries\":[{\"content\":{\"sides\":[{\"content\":{\"connectorIds\":[\"In4\",\"In1\",\"In2\",\"In3\"]},\"type\":\"ConnectorPlacement.EquallySpacedRectSide\",\"uuid\":\"49bdffc0-8e15-4462-b991-b36534669558\"},{\"content\":{\"connectorIds\":[\"Out1\"],\"side\":\"RIGHT\"},\"type\":\"ConnectorPlacement.EquallySpacedRectSide\",\"uuid\":\"379950e5-a8e3-41fb-8f45-c3d731cfbd8a\"},{\"content\":{\"side\":\"TOP\"},\"type\":\"ConnectorPlacement.EquallySpacedRectSide\",\"uuid\":\"38309075-1b62-4fbc-9171-ddac584f70df\"}]},\"type\":\"ConnectorPlacement.EquallySpacedConnector\",\"uuid\":\"335a78c7-f6bb-4aff-a350-269f860e2554\"}],\"packageUris\":[\"http://schema.mathworks.com/mf0/Connector/R2020b\"],\"version\":\"1.0\"}"
  CameraDriver15 : Stateflow chart  TreatAsAtomicUnit=on
      settings: PortSchema="{\"entries\":[{\"content\":{\"sides\":[{\"content\":{\"connectorIds\":[\"In4\",\"In1\",\"In2\",\"In3\"]},\"type\":\"ConnectorPlacement.EquallySpacedRectSide\",\"uuid\":\"49bdffc0-8e15-4462-b991-b36534669558\"},{\"content\":{\"connectorIds\":[\"Out1\"],\"side\":\"RIGHT\"},\"type\":\"ConnectorPlacement.EquallySpacedRectSide\",\"uuid\":\"379950e5-a8e3-41fb-8f45-c3d731cfbd8a\"},{\"content\":{\"side\":\"TOP\"},\"type\":\"ConnectorPlacement.EquallySpacedRectSide\",\"uuid\":\"38309075-1b62-4fbc-9171-ddac584f70df\"}]},\"type\":\"ConnectorPlacement.EquallySpacedConnector\",\"uuid\":\"335a78c7-f6bb-4aff-a350-269f860e2554\"}],\"packageUris\":[\"http://schema.mathworks.com/mf0/Connector/R2020b\"],\"version\":\"1.0\"}"
  CameraDriver16 : Stateflow chart  TreatAsAtomicUnit=on
      settings: PortSchema="{\"entries\":[{\"content\":{\"sides\":[{\"content\":{\"connectorIds\":[\"In4\",\"In1\",\"In2\",\"In3\"]},\"type\":\"ConnectorPlacement.EquallySpacedRectSide\",\"uuid\":\"49bdffc0-8e15-4462-b991-b36534669558\"},{\"content\":{\"connectorIds\":[\"Out1\"],\"side\":\"RIGHT\"},\"type\":\"ConnectorPlacement.EquallySpacedRectSide\",\"uuid\":\"379950e5-a8e3-41fb-8f45-c3d731cfbd8a\"},{\"content\":{\"side\":\"TOP\"},\"type\":\"ConnectorPlacement.EquallySpacedRectSide\",\"uuid\":\"38309075-1b62-4fbc-9171-ddac584f70df\"}]},\"type\":\"ConnectorPlacement.EquallySpacedConnector\",\"uuid\":\"335a78c7-f6bb-4aff-a350-269f860e2554\"}],\"packageUris\":[\"http://schema.mathworks.com/mf0/Connector/R2020b\"],\"version\":\"1.0\"}"
  CameraDriver17 : Stateflow chart  TreatAsAtomicUnit=on
      settings: PortSchema="{\"entries\":[{\"content\":{\"sides\":[{\"content\":{\"connectorIds\":[\"In4\",\"In1\",\"In2\",\"In3\"]},\"type\":\"ConnectorPlacement.EquallySpacedRectSide\",\"uuid\":\"49bdffc0-8e15-4462-b991-b36534669558\"},{\"content\":{\"connectorIds\":[\"Out1\"],\"side\":\"RIGHT\"},\"type\":\"ConnectorPlacement.EquallySpacedRectSide\",\"uuid\":\"379950e5-a8e3-41fb-8f45-c3d731cfbd8a\"},{\"content\":{\"side\":\"TOP\"},\"type\":\"ConnectorPlacement.EquallySpacedRectSide\",\"uuid\":\"38309075-1b62-4fbc-9171-ddac584f70df\"}]},\"type\":\"ConnectorPlacement.EquallySpacedConnector\",\"uuid\":\"335a78c7-f6bb-4aff-a350-269f860e2554\"}],\"packageUris\":[\"http://schema.mathworks.com/mf0/Connector/R2020b\"],\"version\":\"1.0\"}"
  CameraDriver18 : Stateflow chart  TreatAsAtomicUnit=on
      settings: PortSchema="{\"entries\":[{\"content\":{\"sides\":[{\"content\":{\"connectorIds\":[\"In4\",\"In1\",\"In2\",\"In3\"]},\"type\":\"ConnectorPlacement.EquallySpacedRectSide\",\"uuid\":\"49bdffc0-8e15-4462-b991-b36534669558\"},{\"content\":{\"connectorIds\":[\"Out1\"],\"side\":\"RIGHT\"},\"type\":\"ConnectorPlacement.EquallySpacedRectSide\",\"uuid\":\"379950e5-a8e3-41fb-8f45-c3d731cfbd8a\"},{\"content\":{\"side\":\"TOP\"},\"type\":\"ConnectorPlacement.EquallySpacedRectSide\",\"uuid\":\"38309075-1b62-4fbc-9171-ddac584f70df\"}]},\"type\":\"ConnectorPlacement.EquallySpacedConnector\",\"uuid\":\"335a78c7-f6bb-4aff-a350-269f860e2554\"}],\"packageUris\":[\"http://schema.mathworks.com/mf0/Connector/R2020b\"],\"version\":\"1.0\"}"
  CameraDriver19 : Stateflow chart  TreatAsAtomicUnit=on
      settings: PortSchema="{\"entries\":[{\"content\":{\"sides\":[{\"content\":{\"connectorIds\":[\"In4\",\"In1\",\"In2\",\"In3\"]},\"type\":\"ConnectorPlacement.EquallySpacedRectSide\",\"uuid\":\"49bdffc0-8e15-4462-b991-b36534669558\"},{\"content\":{\"connectorIds\":[\"Out1\"],\"side\":\"RIGHT\"},\"type\":\"ConnectorPlacement.EquallySpacedRectSide\",\"uuid\":\"379950e5-a8e3-41fb-8f45-c3d731cfbd8a\"},{\"content\":{\"side\":\"TOP\"},\"type\":\"ConnectorPlacement.EquallySpacedRectSide\",\"uuid\":\"38309075-1b62-4fbc-9171-ddac584f70df\"}]},\"type\":\"ConnectorPlacement.EquallySpacedConnector\",\"uuid\":\"335a78c7-f6bb-4aff-a350-269f860e2554\"}],\"packageUris\":[\"http://schema.mathworks.com/mf0/Connector/R2020b\"],\"version\":\"1.0\"}"
  CameraDriver2 : Stateflow chart  TreatAsAtomicUnit=on
      settings: PortSchema="{\"entries\":[{\"content\":{\"sides\":[{\"content\":{\"connectorIds\":[\"In4\",\"In1\",\"In2\",\"In3\"]},\"type\":\"ConnectorPlacement.EquallySpacedRectSide\",\"uuid\":\"49bdffc0-8e15-4462-b991-b36534669558\"},{\"content\":{\"connectorIds\":[\"Out1\"],\"side\":\"RIGHT\"},\"type\":\"ConnectorPlacement.EquallySpacedRectSide\",\"uuid\":\"379950e5-a8e3-41fb-8f45-c3d731cfbd8a\"},{\"content\":{\"side\":\"TOP\"},\"type\":\"ConnectorPlacement.EquallySpacedRectSide\",\"uuid\":\"38309075-1b62-4fbc-9171-ddac584f70df\"}]},\"type\":\"ConnectorPlacement.EquallySpacedConnector\",\"uuid\":\"335a78c7-f6bb-4aff-a350-269f860e2554\"}],\"packageUris\":[\"http://schema.mathworks.com/mf0/Connector/R2020b\"],\"version\":\"1.0\"}"
  CameraDriver20 : Stateflow chart  TreatAsAtomicUnit=on
      settings: PortSchema="{\"entries\":[{\"content\":{\"sides\":[{\"content\":{\"connectorIds\":[\"In4\",\"In1\",\"In2\",\"In3\"]},\"type\":\"ConnectorPlacement.EquallySpacedRectSide\",\"uuid\":\"49bdffc0-8e15-4462-b991-b36534669558\"},{\"content\":{\"connectorIds\":[\"Out1\"],\"side\":\"RIGHT\"},\"type\":\"ConnectorPlacement.EquallySpacedRectSide\",\"uuid\":\"379950e5-a8e3-41fb-8f45-c3d731cfbd8a\"},{\"content\":{\"side\":\"TOP\"},\"type\":\"ConnectorPlacement.EquallySpacedRectSide\",\"uuid\":\"38309075-1b62-4fbc-9171-ddac584f70df\"}]},\"type\":\"ConnectorPlacement.EquallySpacedConnector\",\"uuid\":\"335a78c7-f6bb-4aff-a350-269f860e2554\"}],\"packageUris\":[\"http://schema.mathworks.com/mf0/Connector/R2020b\"],\"version\":\"1.0\"}"
  CameraDriver21 : Stateflow chart  TreatAsAtomicUnit=on
      settings: PortSchema="{\"entries\":[{\"content\":{\"sides\":[{\"content\":{\"connectorIds\":[\"In4\",\"In1\",\"In2\",\"In3\"]},\"type\":\"ConnectorPlacement.EquallySpacedRectSide\",\"uuid\":\"49bdffc0-8e15-4462-b991-b36534669558\"},{\"content\":{\"connectorIds\":[\"Out1\"],\"side\":\"RIGHT\"},\"type\":\"ConnectorPlacement.EquallySpacedRectSide\",\"uuid\":\"379950e5-a8e3-41fb-8f45-c3d731cfbd8a\"},{\"content\":{\"side\":\"TOP\"},\"type\":\"ConnectorPlacement.EquallySpacedRectSide\",\"uuid\":\"38309075-1b62-4fbc-9171-ddac584f70df\"}]},\"type\":\"ConnectorPlacement.EquallySpacedConnector\",\"uuid\":\"335a78c7-f6bb-4aff-a350-269f860e2554\"}],\"packageUris\":[\"http://schema.mathworks.com/mf0/Connector/R2020b\"],\"version\":\"1.0\"}"
  CameraDriver22 : Stateflow chart  TreatAsAtomicUnit=on
      settings: PortSchema="{\"entries\":[{\"content\":{\"sides\":[{\"content\":{\"connectorIds\":[\"In4\",\"In1\",\"In2\",\"In3\"]},\"type\":\"ConnectorPlacement.EquallySpacedRectSide\",\"uuid\":\"49bdffc0-8e15-4462-b991-b36534669558\"},{\"content\":{\"connectorIds\":[\"Out1\"],\"side\":\"RIGHT\"},\"type\":\"ConnectorPlacement.EquallySpacedRectSide\",\"uuid\":\"379950e5-a8e3-41fb-8f45-c3d731cfbd8a\"},{\"content\":{\"side\":\"TOP\"},\"type\":\"ConnectorPlacement.EquallySpacedRectSide\",\"uuid\":\"38309075-1b62-4fbc-9171-ddac584f70df\"}]},\"type\":\"ConnectorPlacement.EquallySpacedConnector\",\"uuid\":\"335a78c7-f6bb-4aff-a350-269f860e2554\"}],\"packageUris\":[\"http://schema.mathworks.com/mf0/Connector/R2020b\"],\"version\":\"1.0\"}"
  CameraDriver23 : Stateflow chart  TreatAsAtomicUnit=on
      settings: PortSchema="{\"entries\":[{\"content\":{\"sides\":[{\"content\":{\"connectorIds\":[\"In4\",\"In1\",\"In2\",\"In3\"]},\"type\":\"ConnectorPlacement.EquallySpacedRectSide\",\"uuid\":\"49bdffc0-8e15-4462-b991-b36534669558\"},{\"content\":{\"connectorIds\":[\"Out1\"],\"side\":\"RIGHT\"},\"type\":\"ConnectorPlacement.EquallySpacedRectSide\",\"uuid\":\"379950e5-a8e3-41fb-8f45-c3d731cfbd8a\"},{\"content\":{\"side\":\"TOP\"},\"type\":\"ConnectorPlacement.EquallySpacedRectSide\",\"uuid\":\"38309075-1b62-4fbc-9171-ddac584f70df\"}]},\"type\":\"ConnectorPlacement.EquallySpacedConnector\",\"uuid\":\"335a78c7-f6bb-4aff-a350-269f860e2554\"}],\"packageUris\":[\"http://schema.mathworks.com/mf0/Connector/R2020b\"],\"version\":\"1.0\"}"
  CameraDriver24 : Stateflow chart  TreatAsAtomicUnit=on
      settings: PortSchema="{\"entries\":[{\"content\":{\"sides\":[{\"content\":{\"connectorIds\":[\"In4\",\"In1\",\"In2\",\"In3\"]},\"type\":\"ConnectorPlacement.EquallySpacedRectSide\",\"uuid\":\"49bdffc0-8e15-4462-b991-b36534669558\"},{\"content\":{\"connectorIds\":[\"Out1\"],\"side\":\"RIGHT\"},\"type\":\"ConnectorPlacement.EquallySpacedRectSide\",\"uuid\":\"379950e5-a8e3-41fb-8f45-c3d731cfbd8a\"},{\"content\":{\"side\":\"TOP\"},\"type\":\"ConnectorPlacement.EquallySpacedRectSide\",\"uuid\":\"38309075-1b62-4fbc-9171-ddac584f70df\"}]},\"type\":\"ConnectorPlacement.EquallySpacedConnector\",\"uuid\":\"335a78c7-f6bb-4aff-a350-269f860e2554\"}],\"packageUris\":[\"http://schema.mathworks.com/mf0/Connector/R2020b\"],\"version\":\"1.0\"}"
  CameraDriver25 : Stateflow chart  TreatAsAtomicUnit=on
      settings: PortSchema="{\"entries\":[{\"content\":{\"sides\":[{\"content\":{\"connectorIds\":[\"In4\",\"In1\",\"In2\",\"In3\"]},\"type\":\"ConnectorPlacement.EquallySpacedRectSide\",\"uuid\":\"49bdffc0-8e15-4462-b991-b36534669558\"},{\"content\":{\"connectorIds\":[\"Out1\"],\"side\":\"RIGHT\"},\"type\":\"ConnectorPlacement.EquallySpacedRectSide\",\"uuid\":\"379950e5-a8e3-41fb-8f45-c3d731cfbd8a\"},{\"content\":{\"side\":\"TOP\"},\"type\":\"ConnectorPlacement.EquallySpacedRectSide\",\"uuid\":\"38309075-1b62-4fbc-9171-ddac584f70df\"}]},\"type\":\"ConnectorPlacement.EquallySpacedConnector\",\"uuid\":\"335a78c7-f6bb-4aff-a350-269f860e2554\"}],\"packageUris\":[\"http://schema.mathworks.com/mf0/Connector/R2020b\"],\"version\":\"1.0\"}"
  CameraDriver26 : Stateflow chart  TreatAsAtomicUnit=on
      settings: PortSchema="{\"entries\":[{\"content\":{\"sides\":[{\"content\":{\"connectorIds\":[\"In4\",\"In1\",\"In2\",\"In3\"]},\"type\":\"ConnectorPlacement.EquallySpacedRectSide\",\"uuid\":\"49bdffc0-8e15-4462-b991-b36534669558\"},{\"content\":{\"connectorIds\":[\"Out1\"],\"side\":\"RIGHT\"},\"type\":\"ConnectorPlacement.EquallySpacedRectSide\",\"uuid\":\"379950e5-a8e3-41fb-8f45-c3d731cfbd8a\"},{\"content\":{\"side\":\"TOP\"},\"type\":\"ConnectorPlacement.EquallySpacedRectSide\",\"uuid\":\"38309075-1b62-4fbc-9171-ddac584f70df\"}]},\"type\":\"ConnectorPlacement.EquallySpacedConnector\",\"uuid\":\"335a78c7-f6bb-4aff-a350-269f860e2554\"}],\"packageUris\":[\"http://schema.mathworks.com/mf0/Connector/R2020b\"],\"version\":\"1.0\"}"
  CameraDriver27 : Stateflow chart  TreatAsAtomicUnit=on
      settings: PortSchema="{\"entries\":[{\"content\":{\"sides\":[{\"content\":{\"connectorIds\":[\"In4\",\"In1\",\"In2\",\"In3\"]},\"type\":\"ConnectorPlacement.EquallySpacedRectSide\",\"uuid\":\"49bdffc0-8e15-4462-b991-b36534669558\"},{\"content\":{\"connectorIds\":[\"Out1\"],\"side\":\"RIGHT\"},\"type\":\"ConnectorPlacement.EquallySpacedRectSide\",\"uuid\":\"379950e5-a8e3-41fb-8f45-c3d731cfbd8a\"},{\"content\":{\"side\":\"TOP\"},\"type\":\"ConnectorPlacement.EquallySpacedRectSide\",\"uuid\":\"38309075-1b62-4fbc-9171-ddac584f70df\"}]},\"type\":\"ConnectorPlacement.EquallySpacedConnector\",\"uuid\":\"335a78c7-f6bb-4aff-a350-269f860e2554\"}],\"packageUris\":[\"http://schema.mathworks.com/mf0/Connector/R2020b\"],\"version\":\"1.0\"}"
  CameraDriver28 : Stateflow chart  TreatAsAtomicUnit=on
      settings: PortSchema="{\"entries\":[{\"content\":{\"sides\":[{\"content\":{\"connectorIds\":[\"In4\",\"In1\",\"In2\",\"In3\"]},\"type\":\"ConnectorPlacement.EquallySpacedRectSide\",\"uuid\":\"49bdffc0-8e15-4462-b991-b36534669558\"},{\"content\":{\"connectorIds\":[\"Out1\"],\"side\":\"RIGHT\"},\"type\":\"ConnectorPlacement.EquallySpacedRectSide\",\"uuid\":\"379950e5-a8e3-41fb-8f45-c3d731cfbd8a\"},{\"content\":{\"side\":\"TOP\"},\"type\":\"ConnectorPlacement.EquallySpacedRectSide\",\"uuid\":\"38309075-1b62-4fbc-9171-ddac584f70df\"}]},\"type\":\"ConnectorPlacement.EquallySpacedConnector\",\"uuid\":\"335a78c7-f6bb-4aff-a350-269f860e2554\"}],\"packageUris\":[\"http://schema.mathworks.com/mf0/Connector/R2020b\"],\"version\":\"1.0\"}"
  CameraDriver29 : Stateflow chart  TreatAsAtomicUnit=on
      settings: PortSchema="{\"entries\":[{\"content\":{\"sides\":[{\"content\":{\"connectorIds\":[\"In4\",\"In1\",\"In2\",\"In3\"]},\"type\":\"ConnectorPlacement.EquallySpacedRectSide\",\"uuid\":\"49bdffc0-8e15-4462-b991-b36534669558\"},{\"content\":{\"connectorIds\":[\"Out1\"],\"side\":\"RIGHT\"},\"type\":\"ConnectorPlacement.EquallySpacedRectSide\",\"uuid\":\"379950e5-a8e3-41fb-8f45-c3d731cfbd8a\"},{\"content\":{\"side\":\"TOP\"},\"type\":\"ConnectorPlacement.EquallySpacedRectSide\",\"uuid\":\"38309075-1b62-4fbc-9171-ddac584f70df\"}]},\"type\":\"ConnectorPlacement.EquallySpacedConnector\",\"uuid\":\"335a78c7-f6bb-4aff-a350-269f860e2554\"}],\"packageUris\":[\"http://schema.mathworks.com/mf0/Connector/R2020b\"],\"version\":\"1.0\"}"
  CameraDriver3 : Stateflow chart  TreatAsAtomicUnit=on
      settings: PortSchema="{\"entries\":[{\"content\":{\"sides\":[{\"content\":{\"connectorIds\":[\"In4\",\"In1\",\"In2\",\"In3\"]},\"type\":\"ConnectorPlacement.EquallySpacedRectSide\",\"uuid\":\"49bdffc0-8e15-4462-b991-b36534669558\"},{\"content\":{\"connectorIds\":[\"Out1\"],\"side\":\"RIGHT\"},\"type\":\"ConnectorPlacement.EquallySpacedRectSide\",\"uuid\":\"379950e5-a8e3-41fb-8f45-c3d731cfbd8a\"},{\"content\":{\"side\":\"TOP\"},\"type\":\"ConnectorPlacement.EquallySpacedRectSide\",\"uuid\":\"38309075-1b62-4fbc-9171-ddac584f70df\"}]},\"type\":\"ConnectorPlacement.EquallySpacedConnector\",\"uuid\":\"335a78c7-f6bb-4aff-a350-269f860e2554\"}],\"packageUris\":[\"http://schema.mathworks.com/mf0/Connector/R2020b\"],\"version\":\"1.0\"}"
  CameraDriver30 : Stateflow chart  TreatAsAtomicUnit=on
      settings: PortSchema="{\"entries\":[{\"content\":{\"sides\":[{\"content\":{\"connectorIds\":[\"In4\",\"In1\",\"In2\",\"In3\"]},\"type\":\"ConnectorPlacement.EquallySpacedRectSide\",\"uuid\":\"49bdffc0-8e15-4462-b991-b36534669558\"},{\"content\":{\"connectorIds\":[\"Out1\"],\"side\":\"RIGHT\"},\"type\":\"ConnectorPlacement.EquallySpacedRectSide\",\"uuid\":\"379950e5-a8e3-41fb-8f45-c3d731cfbd8a\"},{\"content\":{\"side\":\"TOP\"},\"type\":\"ConnectorPlacement.EquallySpacedRectSide\",\"uuid\":\"38309075-1b62-4fbc-9171-ddac584f70df\"}]},\"type\":\"ConnectorPlacement.EquallySpacedConnector\",\"uuid\":\"335a78c7-f6bb-4aff-a350-269f860e2554\"}],\"packageUris\":[\"http://schema.mathworks.com/mf0/Connector/R2020b\"],\"version\":\"1.0\"}"
  CameraDriver31 : Stateflow chart  TreatAsAtomicUnit=on
      settings: PortSchema="{\"entries\":[{\"content\":{\"sides\":[{\"content\":{\"connectorIds\":[\"In4\",\"In1\",\"In2\",\"In3\"]},\"type\":\"ConnectorPlacement.EquallySpacedRectSide\",\"uuid\":\"49bdffc0-8e15-4462-b991-b36534669558\"},{\"content\":{\"connectorIds\":[\"Out1\"],\"side\":\"RIGHT\"},\"type\":\"ConnectorPlacement.EquallySpacedRectSide\",\"uuid\":\"379950e5-a8e3-41fb-8f45-c3d731cfbd8a\"},{\"content\":{\"side\":\"TOP\"},\"type\":\"ConnectorPlacement.EquallySpacedRectSide\",\"uuid\":\"38309075-1b62-4fbc-9171-ddac584f70df\"}]},\"type\":\"ConnectorPlacement.EquallySpacedConnector\",\"uuid\":\"335a78c7-f6bb-4aff-a350-269f860e2554\"}],\"packageUris\":[\"http://schema.mathworks.com/mf0/Connector/R2020b\"],\"version\":\"1.0\"}"
  CameraDriver4 : Stateflow chart  TreatAsAtomicUnit=on
      settings: PortSchema="{\"entries\":[{\"content\":{\"sides\":[{\"content\":{\"connectorIds\":[\"In4\",\"In1\",\"In2\",\"In3\"]},\"type\":\"ConnectorPlacement.EquallySpacedRectSide\",\"uuid\":\"49bdffc0-8e15-4462-b991-b36534669558\"},{\"content\":{\"connectorIds\":[\"Out1\"],\"side\":\"RIGHT\"},\"type\":\"ConnectorPlacement.EquallySpacedRectSide\",\"uuid\":\"379950e5-a8e3-41fb-8f45-c3d731cfbd8a\"},{\"content\":{\"side\":\"TOP\"},\"type\":\"ConnectorPlacement.EquallySpacedRectSide\",\"uuid\":\"38309075-1b62-4fbc-9171-ddac584f70df\"}]},\"type\":\"ConnectorPlacement.EquallySpacedConnector\",\"uuid\":\"335a78c7-f6bb-4aff-a350-269f860e2554\"}],\"packageUris\":[\"http://schema.mathworks.com/mf0/Connector/R2020b\"],\"version\":\"1.0\"}"
  CameraDriver5 : Stateflow chart  TreatAsAtomicUnit=on
      settings: PortSchema="{\"entries\":[{\"content\":{\"sides\":[{\"content\":{\"connectorIds\":[\"In4\",\"In1\",\"In2\",\"In3\"]},\"type\":\"ConnectorPlacement.EquallySpacedRectSide\",\"uuid\":\"49bdffc0-8e15-4462-b991-b36534669558\"},{\"content\":{\"connectorIds\":[\"Out1\"],\"side\":\"RIGHT\"},\"type\":\"ConnectorPlacement.EquallySpacedRectSide\",\"uuid\":\"379950e5-a8e3-41fb-8f45-c3d731cfbd8a\"},{\"content\":{\"side\":\"TOP\"},\"type\":\"ConnectorPlacement.EquallySpacedRectSide\",\"uuid\":\"38309075-1b62-4fbc-9171-ddac584f70df\"}]},\"type\":\"ConnectorPlacement.EquallySpacedConnector\",\"uuid\":\"335a78c7-f6bb-4aff-a350-269f860e2554\"}],\"packageUris\":[\"http://schema.mathworks.com/mf0/Connector/R2020b\"],\"version\":\"1.0\"}"
  CameraDriver6 : Stateflow chart  TreatAsAtomicUnit=on
      settings: PortSchema="{\"entries\":[{\"content\":{\"sides\":[{\"content\":{\"connectorIds\":[\"In4\",\"In1\",\"In2\",\"In3\"]},\"type\":\"ConnectorPlacement.EquallySpacedRectSide\",\"uuid\":\"49bdffc0-8e15-4462-b991-b36534669558\"},{\"content\":{\"connectorIds\":[\"Out1\"],\"side\":\"RIGHT\"},\"type\":\"ConnectorPlacement.EquallySpacedRectSide\",\"uuid\":\"379950e5-a8e3-41fb-8f45-c3d731cfbd8a\"},{\"content\":{\"side\":\"TOP\"},\"type\":\"ConnectorPlacement.EquallySpacedRectSide\",\"uuid\":\"38309075-1b62-4fbc-9171-ddac584f70df\"}]},\"type\":\"ConnectorPlacement.EquallySpacedConnector\",\"uuid\":\"335a78c7-f6bb-4aff-a350-269f860e2554\"}],\"packageUris\":[\"http://schema.mathworks.com/mf0/Connector/R2020b\"],\"version\":\"1.0\"}"
  CameraDriver7 : Stateflow chart  TreatAsAtomicUnit=on
      settings: PortSchema="{\"entries\":[{\"content\":{\"sides\":[{\"content\":{\"connectorIds\":[\"In4\",\"In1\",\"In2\",\"In3\"]},\"type\":\"ConnectorPlacement.EquallySpacedRectSide\",\"uuid\":\"49bdffc0-8e15-4462-b991-b36534669558\"},{\"content\":{\"connectorIds\":[\"Out1\"],\"side\":\"RIGHT\"},\"type\":\"ConnectorPlacement.EquallySpacedRectSide\",\"uuid\":\"379950e5-a8e3-41fb-8f45-c3d731cfbd8a\"},{\"content\":{\"side\":\"TOP\"},\"type\":\"ConnectorPlacement.EquallySpacedRectSide\",\"uuid\":\"38309075-1b62-4fbc-9171-ddac584f70df\"}]},\"type\":\"ConnectorPlacement.EquallySpacedConnector\",\"uuid\":\"335a78c7-f6bb-4aff-a350-269f860e2554\"}],\"packageUris\":[\"http://schema.mathworks.com/mf0/Connector/R2020b\"],\"version\":\"1.0\"}"
  CameraDriver8 : Stateflow chart  TreatAsAtomicUnit=on
      settings: PortSchema="{\"entries\":[{\"content\":{\"sides\":[{\"content\":{\"connectorIds\":[\"In4\",\"In1\",\"In2\",\"In3\"]},\"type\":\"ConnectorPlacement.EquallySpacedRectSide\",\"uuid\":\"49bdffc0-8e15-4462-b991-b36534669558\"},{\"content\":{\"connectorIds\":[\"Out1\"],\"side\":\"RIGHT\"},\"type\":\"ConnectorPlacement.EquallySpacedRectSide\",\"uuid\":\"379950e5-a8e3-41fb-8f45-c3d731cfbd8a\"},{\"content\":{\"side\":\"TOP\"},\"type\":\"ConnectorPlacement.EquallySpacedRectSide\",\"uuid\":\"38309075-1b62-4fbc-9171-ddac584f70df\"}]},\"type\":\"ConnectorPlacement.EquallySpacedConnector\",\"uuid\":\"335a78c7-f6bb-4aff-a350-269f860e2554\"}],\"packageUris\":[\"http://schema.mathworks.com/mf0/Connector/R2020b\"],\"version\":\"1.0\"}"
  CameraDriver9 : Stateflow chart  TreatAsAtomicUnit=on
      settings: PortSchema="{\"entries\":[{\"content\":{\"sides\":[{\"content\":{\"connectorIds\":[\"In4\",\"In1\",\"In2\",\"In3\"]},\"type\":\"ConnectorPlacement.EquallySpacedRectSide\",\"uuid\":\"49bdffc0-8e15-4462-b991-b36534669558\"},{\"content\":{\"connectorIds\":[\"Out1\"],\"side\":\"RIGHT\"},\"type\":\"ConnectorPlacement.EquallySpacedRectSide\",\"uuid\":\"379950e5-a8e3-41fb-8f45-c3d731cfbd8a\"},{\"content\":{\"side\":\"TOP\"},\"type\":\"ConnectorPlacement.EquallySpacedRectSide\",\"uuid\":\"38309075-1b62-4fbc-9171-ddac584f70df\"}]},\"type\":\"ConnectorPlacement.EquallySpacedConnector\",\"uuid\":\"335a78c7-f6bb-4aff-a350-269f860e2554\"}],\"packageUris\":[\"http://schema.mathworks.com/mf0/Connector/R2020b\"],\"version\":\"1.0\"}"
  CameraScheduler : Stateflow chart  TreatAsAtomicUnit=on
      settings: PortSchema="{\"entries\":[{\"content\":{\"sides\":[{\"content\":{\"connectorIds\":[\"In1\"]},\"type\":\"ConnectorPlacement.EquallySpacedRectSide\",\"uuid\":\"228150a7-62a2-46d0-a1ac-a8e868d835b5\"},{\"content\":{\"connectorIds\":[\"Out2\",\"Out3\",\"Out1\"],\"side\":\"RIGHT\"},\"type\":\"ConnectorPlacement.EquallySpacedRectSide\",\"uuid\":\"cb1c6840-c5bf-4913-92c2-1c054d368f87\"},{\"content\":{\"side\":\"TOP\"},\"type\":\"ConnectorPlacement.EquallySpacedRectSide\",\"uuid\":\"3633cd87-b3f9-48c9-80b7-73d7f17aa7ad\"}]},\"type\":\"ConnectorPlacement.EquallySpacedConnector\",\"uuid\":\"2553d532-cb7a-499b-b98c-b91f81677a07\"}],\"packageUris\":[\"http://schema.mathworks.com/mf0/Connector/R2020b\"],\"version\":\"1.0\"}"
  CameraScheduler1 : Stateflow chart  TreatAsAtomicUnit=on
      settings: PortSchema="{\"entries\":[{\"content\":{\"sides\":[{\"content\":{\"connectorIds\":[\"In1\"]},\"type\":\"ConnectorPlacement.EquallySpacedRectSide\",\"uuid\":\"335362b2-4c4f-40e6-baf0-d287f6971824\"},{\"content\":{\"connectorIds\":[\"Out2\",\"Out1\"],\"side\":\"RIGHT\"},\"type\":\"ConnectorPlacement.EquallySpacedRectSide\",\"uuid\":\"7ee54d08-aa3e-4d6f-8253-6f749626479a\"},{\"content\":{\"side\":\"TOP\"},\"type\":\"ConnectorPlacement.EquallySpacedRectSide\",\"uuid\":\"7bf47310-47f4-4483-b0d1-b8a087b66b77\"}]},\"type\":\"ConnectorPlacement.EquallySpacedConnector\",\"uuid\":\"fb61df21-9632-41f0-9cfa-ce5060944b6c\"}],\"packageUris\":[\"http://schema.mathworks.com/mf0/Connector/R2020b\"],\"version\":\"1.0\"}"
  CameraScheduler10 : Stateflow chart  TreatAsAtomicUnit=on
      settings: PortSchema="{\"entries\":[{\"content\":{\"sides\":[{\"content\":{\"connectorIds\":[\"In1\"]},\"type\":\"ConnectorPlacement.EquallySpacedRectSide\",\"uuid\":\"228150a7-62a2-46d0-a1ac-a8e868d835b5\"},{\"content\":{\"connectorIds\":[\"Out2\",\"Out1\"],\"side\":\"RIGHT\"},\"type\":\"ConnectorPlacement.EquallySpacedRectSide\",\"uuid\":\"cb1c6840-c5bf-4913-92c2-1c054d368f87\"},{\"content\":{\"side\":\"TOP\"},\"type\":\"ConnectorPlacement.EquallySpacedRectSide\",\"uuid\":\"3633cd87-b3f9-48c9-80b7-73d7f17aa7ad\"}]},\"type\":\"ConnectorPlacement.EquallySpacedConnector\",\"uuid\":\"2553d532-cb7a-499b-b98c-b91f81677a07\"}],\"packageUris\":[\"http://schema.mathworks.com/mf0/Connector/R2020b\"],\"version\":\"1.0\"}"
  CameraScheduler11 : Stateflow chart  TreatAsAtomicUnit=on
      settings: PortSchema="{\"entries\":[{\"content\":{\"sides\":[{\"content\":{\"connectorIds\":[\"In1\"]},\"type\":\"ConnectorPlacement.EquallySpacedRectSide\",\"uuid\":\"335362b2-4c4f-40e6-baf0-d287f6971824\"},{\"content\":{\"connectorIds\":[\"Out2\",\"Out1\"],\"side\":\"RIGHT\"},\"type\":\"ConnectorPlacement.EquallySpacedRectSide\",\"uuid\":\"7ee54d08-aa3e-4d6f-8253-6f749626479a\"},{\"content\":{\"side\":\"TOP\"},\"type\":\"ConnectorPlacement.EquallySpacedRectSide\",\"uuid\":\"7bf47310-47f4-4483-b0d1-b8a087b66b77\"}]},\"type\":\"ConnectorPlacement.EquallySpacedConnector\",\"uuid\":\"fb61df21-9632-41f0-9cfa-ce5060944b6c\"}],\"packageUris\":[\"http://schema.mathworks.com/mf0/Connector/R2020b\"],\"version\":\"1.0\"}"
  CameraScheduler12 : Stateflow chart  TreatAsAtomicUnit=on
      settings: PortSchema="{\"entries\":[{\"content\":{\"sides\":[{\"content\":{\"connectorIds\":[\"In1\"]},\"type\":\"ConnectorPlacement.EquallySpacedRectSide\",\"uuid\":\"228150a7-62a2-46d0-a1ac-a8e868d835b5\"},{\"content\":{\"connectorIds\":[\"Out2\",\"Out1\"],\"side\":\"RIGHT\"},\"type\":\"ConnectorPlacement.EquallySpacedRectSide\",\"uuid\":\"cb1c6840-c5bf-4913-92c2-1c054d368f87\"},{\"content\":{\"side\":\"TOP\"},\"type\":\"ConnectorPlacement.EquallySpacedRectSide\",\"uuid\":\"3633cd87-b3f9-48c9-80b7-73d7f17aa7ad\"}]},\"type\":\"ConnectorPlacement.EquallySpacedConnector\",\"uuid\":\"2553d532-cb7a-499b-b98c-b91f81677a07\"}],\"packageUris\":[\"http://schema.mathworks.com/mf0/Connector/R2020b\"],\"version\":\"1.0\"}"
  CameraScheduler13 : Stateflow chart  TreatAsAtomicUnit=on
      settings: PortSchema="{\"entries\":[{\"content\":{\"sides\":[{\"content\":{\"connectorIds\":[\"In1\"]},\"type\":\"ConnectorPlacement.EquallySpacedRectSide\",\"uuid\":\"335362b2-4c4f-40e6-baf0-d287f6971824\"},{\"content\":{\"connectorIds\":[\"Out2\",\"Out1\"],\"side\":\"RIGHT\"},\"type\":\"ConnectorPlacement.EquallySpacedRectSide\",\"uuid\":\"7ee54d08-aa3e-4d6f-8253-6f749626479a\"},{\"content\":{\"side\":\"TOP\"},\"type\":\"ConnectorPlacement.EquallySpacedRectSide\",\"uuid\":\"7bf47310-47f4-4483-b0d1-b8a087b66b77\"}]},\"type\":\"ConnectorPlacement.EquallySpacedConnector\",\"uuid\":\"fb61df21-9632-41f0-9cfa-ce5060944b6c\"}],\"packageUris\":[\"http://schema.mathworks.com/mf0/Connector/R2020b\"],\"version\":\"1.0\"}"
  CameraScheduler14 : Stateflow chart  TreatAsAtomicUnit=on
      settings: PortSchema="{\"entries\":[{\"content\":{\"sides\":[{\"content\":{\"connectorIds\":[\"In1\"]},\"type\":\"ConnectorPlacement.EquallySpacedRectSide\",\"uuid\":\"228150a7-62a2-46d0-a1ac-a8e868d835b5\"},{\"content\":{\"connectorIds\":[\"Out2\",\"Out1\"],\"side\":\"RIGHT\"},\"type\":\"ConnectorPlacement.EquallySpacedRectSide\",\"uuid\":\"cb1c6840-c5bf-4913-92c2-1c054d368f87\"},{\"content\":{\"side\":\"TOP\"},\"type\":\"ConnectorPlacement.EquallySpacedRectSide\",\"uuid\":\"3633cd87-b3f9-48c9-80b7-73d7f17aa7ad\"}]},\"type\":\"ConnectorPlacement.EquallySpacedConnector\",\"uuid\":\"2553d532-cb7a-499b-b98c-b91f81677a07\"}],\"packageUris\":[\"http://schema.mathworks.com/mf0/Connector/R2020b\"],\"version\":\"1.0\"}"
  CameraScheduler15 : Stateflow chart  TreatAsAtomicUnit=on
      settings: PortSchema="{\"entries\":[{\"content\":{\"sides\":[{\"content\":{\"connectorIds\":[\"In1\"]},\"type\":\"ConnectorPlacement.EquallySpacedRectSide\",\"uuid\":\"335362b2-4c4f-40e6-baf0-d287f6971824\"},{\"content\":{\"connectorIds\":[\"Out2\",\"Out1\"],\"side\":\"RIGHT\"},\"type\":\"ConnectorPlacement.EquallySpacedRectSide\",\"uuid\":\"7ee54d08-aa3e-4d6f-8253-6f749626479a\"},{\"content\":{\"side\":\"TOP\"},\"type\":\"ConnectorPlacement.EquallySpacedRectSide\",\"uuid\":\"7bf47310-47f4-4483-b0d1-b8a087b66b77\"}]},\"type\":\"ConnectorPlacement.EquallySpacedConnector\",\"uuid\":\"fb61df21-9632-41f0-9cfa-ce5060944b6c\"}],\"packageUris\":[\"http://schema.mathworks.com/mf0/Connector/R2020b\"],\"version\":\"1.0\"}"
  CameraScheduler16 : Stateflow chart  TreatAsAtomicUnit=on
      settings: PortSchema="{\"entries\":[{\"content\":{\"sides\":[{\"content\":{\"connectorIds\":[\"In1\"]},\"type\":\"ConnectorPlacement.EquallySpacedRectSide\",\"uuid\":\"228150a7-62a2-46d0-a1ac-a8e868d835b5\"},{\"content\":{\"connectorIds\":[\"Out2\",\"Out3\",\"Out1\"],\"side\":\"RIGHT\"},\"type\":\"ConnectorPlacement.EquallySpacedRectSide\",\"uuid\":\"cb1c6840-c5bf-4913-92c2-1c054d368f87\"},{\"content\":{\"side\":\"TOP\"},\"type\":\"ConnectorPlacement.EquallySpacedRectSide\",\"uuid\":\"3633cd87-b3f9-48c9-80b7-73d7f17aa7ad\"}]},\"type\":\"ConnectorPlacement.EquallySpacedConnector\",\"uuid\":\"2553d532-cb7a-499b-b98c-b91f81677a07\"}],\"packageUris\":[\"http://schema.mathworks.com/mf0/Connector/R2020b\"],\"version\":\"1.0\"}"
  CameraScheduler17 : Stateflow chart  TreatAsAtomicUnit=on
      settings: PortSchema="{\"entries\":[{\"content\":{\"sides\":[{\"content\":{\"connectorIds\":[\"In1\"]},\"type\":\"ConnectorPlacement.EquallySpacedRectSide\",\"uuid\":\"335362b2-4c4f-40e6-baf0-d287f6971824\"},{\"content\":{\"connectorIds\":[\"Out2\",\"Out1\"],\"side\":\"RIGHT\"},\"type\":\"ConnectorPlacement.EquallySpacedRectSide\",\"uuid\":\"7ee54d08-aa3e-4d6f-8253-6f749626479a\"},{\"content\":{\"side\":\"TOP\"},\"type\":\"ConnectorPlacement.EquallySpacedRectSide\",\"uuid\":\"7bf47310-47f4-4483-b0d1-b8a087b66b77\"}]},\"type\":\"ConnectorPlacement.EquallySpacedConnector\",\"uuid\":\"fb61df21-9632-41f0-9cfa-ce5060944b6c\"}],\"packageUris\":[\"http://schema.mathworks.com/mf0/Connector/R2020b\"],\"version\":\"1.0\"}"
  CameraScheduler18 : Stateflow chart  TreatAsAtomicUnit=on
      settings: PortSchema="{\"entries\":[{\"content\":{\"sides\":[{\"content\":{\"connectorIds\":[\"In1\"]},\"type\":\"ConnectorPlacement.EquallySpacedRectSide\",\"uuid\":\"228150a7-62a2-46d0-a1ac-a8e868d835b5\"},{\"content\":{\"connectorIds\":[\"Out2\",\"Out1\"],\"side\":\"RIGHT\"},\"type\":\"ConnectorPlacement.EquallySpacedRectSide\",\"uuid\":\"cb1c6840-c5bf-4913-92c2-1c054d368f87\"},{\"content\":{\"side\":\"TOP\"},\"type\":\"ConnectorPlacement.EquallySpacedRectSide\",\"uuid\":\"3633cd87-b3f9-48c9-80b7-73d7f17aa7ad\"}]},\"type\":\"ConnectorPlacement.EquallySpacedConnector\",\"uuid\":\"2553d532-cb7a-499b-b98c-b91f81677a07\"}],\"packageUris\":[\"http://schema.mathworks.com/mf0/Connector/R2020b\"],\"version\":\"1.0\"}"
  CameraScheduler19 : Stateflow chart  TreatAsAtomicUnit=on
      settings: PortSchema="{\"entries\":[{\"content\":{\"sides\":[{\"content\":{\"connectorIds\":[\"In1\"]},\"type\":\"ConnectorPlacement.EquallySpacedRectSide\",\"uuid\":\"335362b2-4c4f-40e6-baf0-d287f6971824\"},{\"content\":{\"connectorIds\":[\"Out2\",\"Out1\"],\"side\":\"RIGHT\"},\"type\":\"ConnectorPlacement.EquallySpacedRectSide\",\"uuid\":\"7ee54d08-aa3e-4d6f-8253-6f749626479a\"},{\"content\":{\"side\":\"TOP\"},\"type\":\"ConnectorPlacement.EquallySpacedRectSide\",\"uuid\":\"7bf47310-47f4-4483-b0d1-b8a087b66b77\"}]},\"type\":\"ConnectorPlacement.EquallySpacedConnector\",\"uuid\":\"fb61df21-9632-41f0-9cfa-ce5060944b6c\"}],\"packageUris\":[\"http://schema.mathworks.com/mf0/Connector/R2020b\"],\"version\":\"1.0\"}"
  CameraScheduler2 : Stateflow chart  TreatAsAtomicUnit=on
      settings: PortSchema="{\"entries\":[{\"content\":{\"sides\":[{\"content\":{\"connectorIds\":[\"In1\"]},\"type\":\"ConnectorPlacement.EquallySpacedRectSide\",\"uuid\":\"228150a7-62a2-46d0-a1ac-a8e868d835b5\"},{\"content\":{\"connectorIds\":[\"Out2\",\"Out3\",\"Out1\"],\"side\":\"RIGHT\"},\"type\":\"ConnectorPlacement.EquallySpacedRectSide\",\"uuid\":\"cb1c6840-c5bf-4913-92c2-1c054d368f87\"},{\"content\":{\"side\":\"TOP\"},\"type\":\"ConnectorPlacement.EquallySpacedRectSide\",\"uuid\":\"3633cd87-b3f9-48c9-80b7-73d7f17aa7ad\"}]},\"type\":\"ConnectorPlacement.EquallySpacedConnector\",\"uuid\":\"2553d532-cb7a-499b-b98c-b91f81677a07\"}],\"packageUris\":[\"http://schema.mathworks.com/mf0/Connector/R2020b\"],\"version\":\"1.0\"}"
  CameraScheduler20 : Stateflow chart  TreatAsAtomicUnit=on
      settings: PortSchema="{\"entries\":[{\"content\":{\"sides\":[{\"content\":{\"connectorIds\":[\"In1\"]},\"type\":\"ConnectorPlacement.EquallySpacedRectSide\",\"uuid\":\"228150a7-62a2-46d0-a1ac-a8e868d835b5\"},{\"content\":{\"connectorIds\":[\"Out2\",\"Out1\"],\"side\":\"RIGHT\"},\"type\":\"ConnectorPlacement.EquallySpacedRectSide\",\"uuid\":\"cb1c6840-c5bf-4913-92c2-1c054d368f87\"},{\"content\":{\"side\":\"TOP\"},\"type\":\"ConnectorPlacement.EquallySpacedRectSide\",\"uuid\":\"3633cd87-b3f9-48c9-80b7-73d7f17aa7ad\"}]},\"type\":\"ConnectorPlacement.EquallySpacedConnector\",\"uuid\":\"2553d532-cb7a-499b-b98c-b91f81677a07\"}],\"packageUris\":[\"http://schema.mathworks.com/mf0/Connector/R2020b\"],\"version\":\"1.0\"}"
  CameraScheduler21 : Stateflow chart  TreatAsAtomicUnit=on
      settings: PortSchema="{\"entries\":[{\"content\":{\"sides\":[{\"content\":{\"connectorIds\":[\"In1\"]},\"type\":\"ConnectorPlacement.EquallySpacedRectSide\",\"uuid\":\"335362b2-4c4f-40e6-baf0-d287f6971824\"},{\"content\":{\"connectorIds\":[\"Out2\",\"Out1\"],\"side\":\"RIGHT\"},\"type\":\"ConnectorPlacement.EquallySpacedRectSide\",\"uuid\":\"7ee54d08-aa3e-4d6f-8253-6f749626479a\"},{\"content\":{\"side\":\"TOP\"},\"type\":\"ConnectorPlacement.EquallySpacedRectSide\",\"uuid\":\"7bf47310-47f4-4483-b0d1-b8a087b66b77\"}]},\"type\":\"ConnectorPlacement.EquallySpacedConnector\",\"uuid\":\"fb61df21-9632-41f0-9cfa-ce5060944b6c\"}],\"packageUris\":[\"http://schema.mathworks.com/mf0/Connector/R2020b\"],\"version\":\"1.0\"}"
  CameraScheduler22 : Stateflow chart  TreatAsAtomicUnit=on
      settings: PortSchema="{\"entries\":[{\"content\":{\"sides\":[{\"content\":{\"connectorIds\":[\"In1\"]},\"type\":\"ConnectorPlacement.EquallySpacedRectSide\",\"uuid\":\"228150a7-62a2-46d0-a1ac-a8e868d835b5\"},{\"content\":{\"connectorIds\":[\"Out2\",\"Out1\"],\"side\":\"RIGHT\"},\"type\":\"ConnectorPlacement.EquallySpacedRectSide\",\"uuid\":\"cb1c6840-c5bf-4913-92c2-1c054d368f87\"},{\"content\":{\"side\":\"TOP\"},\"type\":\"ConnectorPlacement.EquallySpacedRectSide\",\"uuid\":\"3633cd87-b3f9-48c9-80b7-73d7f17aa7ad\"}]},\"type\":\"ConnectorPlacement.EquallySpacedConnector\",\"uuid\":\"2553d532-cb7a-499b-b98c-b91f81677a07\"}],\"packageUris\":[\"http://schema.mathworks.com/mf0/Connector/R2020b\"],\"version\":\"1.0\"}"
  CameraScheduler23 : Stateflow chart  TreatAsAtomicUnit=on
      settings: PortSchema="{\"entries\":[{\"content\":{\"sides\":[{\"content\":{\"connectorIds\":[\"In1\"]},\"type\":\"ConnectorPlacement.EquallySpacedRectSide\",\"uuid\":\"335362b2-4c4f-40e6-baf0-d287f6971824\"},{\"content\":{\"connectorIds\":[\"Out2\",\"Out1\"],\"side\":\"RIGHT\"},\"type\":\"ConnectorPlacement.EquallySpacedRectSide\",\"uuid\":\"7ee54d08-aa3e-4d6f-8253-6f749626479a\"},{\"content\":{\"side\":\"TOP\"},\"type\":\"ConnectorPlacement.EquallySpacedRectSide\",\"uuid\":\"7bf47310-47f4-4483-b0d1-b8a087b66b77\"}]},\"type\":\"ConnectorPlacement.EquallySpacedConnector\",\"uuid\":\"fb61df21-9632-41f0-9cfa-ce5060944b6c\"}],\"packageUris\":[\"http://schema.mathworks.com/mf0/Connector/R2020b\"],\"version\":\"1.0\"}"
  CameraScheduler24 : Stateflow chart  TreatAsAtomicUnit=on
      settings: PortSchema="{\"entries\":[{\"content\":{\"sides\":[{\"content\":{\"connectorIds\":[\"In1\"]},\"type\":\"ConnectorPlacement.EquallySpacedRectSide\",\"uuid\":\"228150a7-62a2-46d0-a1ac-a8e868d835b5\"},{\"content\":{\"connectorIds\":[\"Out2\",\"Out3\",\"Out1\"],\"side\":\"RIGHT\"},\"type\":\"ConnectorPlacement.EquallySpacedRectSide\",\"uuid\":\"cb1c6840-c5bf-4913-92c2-1c054d368f87\"},{\"content\":{\"side\":\"TOP\"},\"type\":\"ConnectorPlacement.EquallySpacedRectSide\",\"uuid\":\"3633cd87-b3f9-48c9-80b7-73d7f17aa7ad\"}]},\"type\":\"ConnectorPlacement.EquallySpacedConnector\",\"uuid\":\"2553d532-cb7a-499b-b98c-b91f81677a07\"}],\"packageUris\":[\"http://schema.mathworks.com/mf0/Connector/R2020b\"],\"version\":\"1.0\"}"
  CameraScheduler25 : Stateflow chart  TreatAsAtomicUnit=on
      settings: PortSchema="{\"entries\":[{\"content\":{\"sides\":[{\"content\":{\"connectorIds\":[\"In1\"]},\"type\":\"ConnectorPlacement.EquallySpacedRectSide\",\"uuid\":\"335362b2-4c4f-40e6-baf0-d287f6971824\"},{\"content\":{\"connectorIds\":[\"Out2\",\"Out1\"],\"side\":\"RIGHT\"},\"type\":\"ConnectorPlacement.EquallySpacedRectSide\",\"uuid\":\"7ee54d08-aa3e-4d6f-8253-6f749626479a\"},{\"content\":{\"side\":\"TOP\"},\"type\":\"ConnectorPlacement.EquallySpacedRectSide\",\"uuid\":\"7bf47310-47f4-4483-b0d1-b8a087b66b77\"}]},\"type\":\"ConnectorPlacement.EquallySpacedConnector\",\"uuid\":\"fb61df21-9632-41f0-9cfa-ce5060944b6c\"}],\"packageUris\":[\"http://schema.mathworks.com/mf0/Connector/R2020b\"],\"version\":\"1.0\"}"
  CameraScheduler26 : Stateflow chart  TreatAsAtomicUnit=on
      settings: PortSchema="{\"entries\":[{\"content\":{\"sides\":[{\"content\":{\"connectorIds\":[\"In1\"]},\"type\":\"ConnectorPlacement.EquallySpacedRectSide\",\"uuid\":\"228150a7-62a2-46d0-a1ac-a8e868d835b5\"},{\"content\":{\"connectorIds\":[\"Out2\",\"Out3\",\"Out1\"],\"side\":\"RIGHT\"},\"type\":\"ConnectorPlacement.EquallySpacedRectSide\",\"uuid\":\"cb1c6840-c5bf-4913-92c2-1c054d368f87\"},{\"content\":{\"side\":\"TOP\"},\"type\":\"ConnectorPlacement.EquallySpacedRectSide\",\"uuid\":\"3633cd87-b3f9-48c9-80b7-73d7f17aa7ad\"}]},\"type\":\"ConnectorPlacement.EquallySpacedConnector\",\"uuid\":\"2553d532-cb7a-499b-b98c-b91f81677a07\"}],\"packageUris\":[\"http://schema.mathworks.com/mf0/Connector/R2020b\"],\"version\":\"1.0\"}"
  CameraScheduler27 : Stateflow chart  TreatAsAtomicUnit=on
      settings: PortSchema="{\"entries\":[{\"content\":{\"sides\":[{\"content\":{\"connectorIds\":[\"In1\"]},\"type\":\"ConnectorPlacement.EquallySpacedRectSide\",\"uuid\":\"335362b2-4c4f-40e6-baf0-d287f6971824\"},{\"content\":{\"connectorIds\":[\"Out2\",\"Out1\"],\"side\":\"RIGHT\"},\"type\":\"ConnectorPlacement.EquallySpacedRectSide\",\"uuid\":\"7ee54d08-aa3e-4d6f-8253-6f749626479a\"},{\"content\":{\"side\":\"TOP\"},\"type\":\"ConnectorPlacement.EquallySpacedRectSide\",\"uuid\":\"7bf47310-47f4-4483-b0d1-b8a087b66b77\"}]},\"type\":\"ConnectorPlacement.EquallySpacedConnector\",\"uuid\":\"fb61df21-9632-41f0-9cfa-ce5060944b6c\"}],\"packageUris\":[\"http://schema.mathworks.com/mf0/Connector/R2020b\"],\"version\":\"1.0\"}"
  CameraScheduler28 : Stateflow chart  TreatAsAtomicUnit=on
      settings: PortSchema="{\"entries\":[{\"content\":{\"sides\":[{\"content\":{\"connectorIds\":[\"In1\"]},\"type\":\"ConnectorPlacement.EquallySpacedRectSide\",\"uuid\":\"228150a7-62a2-46d0-a1ac-a8e868d835b5\"},{\"content\":{\"connectorIds\":[\"Out2\",\"Out3\",\"Out1\"],\"side\":\"RIGHT\"},\"type\":\"ConnectorPlacement.EquallySpacedRectSide\",\"uuid\":\"cb1c6840-c5bf-4913-92c2-1c054d368f87\"},{\"content\":{\"side\":\"TOP\"},\"type\":\"ConnectorPlacement.EquallySpacedRectSide\",\"uuid\":\"3633cd87-b3f9-48c9-80b7-73d7f17aa7ad\"}]},\"type\":\"ConnectorPlacement.EquallySpacedConnector\",\"uuid\":\"2553d532-cb7a-499b-b98c-b91f81677a07\"}],\"packageUris\":[\"http://schema.mathworks.com/mf0/Connector/R2020b\"],\"version\":\"1.0\"}"
  CameraScheduler29 : Stateflow chart  TreatAsAtomicUnit=on
      settings: PortSchema="{\"entries\":[{\"content\":{\"sides\":[{\"content\":{\"connectorIds\":[\"In1\"]},\"type\":\"ConnectorPlacement.EquallySpacedRectSide\",\"uuid\":\"335362b2-4c4f-40e6-baf0-d287f6971824\"},{\"content\":{\"connectorIds\":[\"Out2\",\"Out1\"],\"side\":\"RIGHT\"},\"type\":\"ConnectorPlacement.EquallySpacedRectSide\",\"uuid\":\"7ee54d08-aa3e-4d6f-8253-6f749626479a\"},{\"content\":{\"side\":\"TOP\"},\"type\":\"ConnectorPlacement.EquallySpacedRectSide\",\"uuid\":\"7bf47310-47f4-4483-b0d1-b8a087b66b77\"}]},\"type\":\"ConnectorPlacement.EquallySpacedConnector\",\"uuid\":\"fb61df21-9632-41f0-9cfa-ce5060944b6c\"}],\"packageUris\":[\"http://schema.mathworks.com/mf0/Connector/R2020b\"],\"version\":\"1.0\"}"
  CameraScheduler3 : Stateflow chart  TreatAsAtomicUnit=on
      settings: PortSchema="{\"entries\":[{\"content\":{\"sides\":[{\"content\":{\"connectorIds\":[\"In1\"]},\"type\":\"ConnectorPlacement.EquallySpacedRectSide\",\"uuid\":\"335362b2-4c4f-40e6-baf0-d287f6971824\"},{\"content\":{\"connectorIds\":[\"Out2\",\"Out1\"],\"side\":\"RIGHT\"},\"type\":\"ConnectorPlacement.EquallySpacedRectSide\",\"uuid\":\"7ee54d08-aa3e-4d6f-8253-6f749626479a\"},{\"content\":{\"side\":\"TOP\"},\"type\":\"ConnectorPlacement.EquallySpacedRectSide\",\"uuid\":\"7bf47310-47f4-4483-b0d1-b8a087b66b77\"}]},\"type\":\"ConnectorPlacement.EquallySpacedConnector\",\"uuid\":\"fb61df21-9632-41f0-9cfa-ce5060944b6c\"}],\"packageUris\":[\"http://schema.mathworks.com/mf0/Connector/R2020b\"],\"version\":\"1.0\"}"
  CameraScheduler30 : Stateflow chart  TreatAsAtomicUnit=on
      settings: PortSchema="{\"entries\":[{\"content\":{\"sides\":[{\"content\":{\"connectorIds\":[\"In1\"]},\"type\":\"ConnectorPlacement.EquallySpacedRectSide\",\"uuid\":\"228150a7-62a2-46d0-a1ac-a8e868d835b5\"},{\"content\":{\"connectorIds\":[\"Out2\",\"Out1\"],\"side\":\"RIGHT\"},\"type\":\"ConnectorPlacement.EquallySpacedRectSide\",\"uuid\":\"cb1c6840-c5bf-4913-92c2-1c054d368f87\"},{\"content\":{\"side\":\"TOP\"},\"type\":\"ConnectorPlacement.EquallySpacedRectSide\",\"uuid\":\"3633cd87-b3f9-48c9-80b7-73d7f17aa7ad\"}]},\"type\":\"ConnectorPlacement.EquallySpacedConnector\",\"uuid\":\"2553d532-cb7a-499b-b98c-b91f81677a07\"}],\"packageUris\":[\"http://schema.mathworks.com/mf0/Connector/R2020b\"],\"version\":\"1.0\"}"
  CameraScheduler31 : Stateflow chart  TreatAsAtomicUnit=on
      settings: PortSchema="{\"entries\":[{\"content\":{\"sides\":[{\"content\":{\"connectorIds\":[\"In1\"]},\"type\":\"ConnectorPlacement.EquallySpacedRectSide\",\"uuid\":\"335362b2-4c4f-40e6-baf0-d287f6971824\"},{\"content\":{\"connectorIds\":[\"Out2\",\"Out1\"],\"side\":\"RIGHT\"},\"type\":\"ConnectorPlacement.EquallySpacedRectSide\",\"uuid\":\"7ee54d08-aa3e-4d6f-8253-6f749626479a\"},{\"content\":{\"side\":\"TOP\"},\"type\":\"ConnectorPlacement.EquallySpacedRectSide\",\"uuid\":\"7bf47310-47f4-4483-b0d1-b8a087b66b77\"}]},\"type\":\"ConnectorPlacement.EquallySpacedConnector\",\"uuid\":\"fb61df21-9632-41f0-9cfa-ce5060944b6c\"}],\"packageUris\":[\"http://schema.mathworks.com/mf0/Connector/R2020b\"],\"version\":\"1.0\"}"
  CameraScheduler4 : Stateflow chart  TreatAsAtomicUnit=on
      settings: PortSchema="{\"entries\":[{\"content\":{\"sides\":[{\"content\":{\"connectorIds\":[\"In1\"]},\"type\":\"ConnectorPlacement.EquallySpacedRectSide\",\"uuid\":\"228150a7-62a2-46d0-a1ac-a8e868d835b5\"},{\"content\":{\"connectorIds\":[\"Out2\",\"Out3\",\"Out1\"],\"side\":\"RIGHT\"},\"type\":\"ConnectorPlacement.EquallySpacedRectSide\",\"uuid\":\"cb1c6840-c5bf-4913-92c2-1c054d368f87\"},{\"content\":{\"side\":\"TOP\"},\"type\":\"ConnectorPlacement.EquallySpacedRectSide\",\"uuid\":\"3633cd87-b3f9-48c9-80b7-73d7f17aa7ad\"}]},\"type\":\"ConnectorPlacement.EquallySpacedConnector\",\"uuid\":\"2553d532-cb7a-499b-b98c-b91f81677a07\"}],\"packageUris\":[\"http://schema.mathworks.com/mf0/Connector/R2020b\"],\"version\":\"1.0\"}"
  CameraScheduler5 : Stateflow chart  TreatAsAtomicUnit=on
      settings: PortSchema="{\"entries\":[{\"content\":{\"sides\":[{\"content\":{\"connectorIds\":[\"In1\"]},\"type\":\"ConnectorPlacement.EquallySpacedRectSide\",\"uuid\":\"335362b2-4c4f-40e6-baf0-d287f6971824\"},{\"content\":{\"connectorIds\":[\"Out2\",\"Out1\"],\"side\":\"RIGHT\"},\"type\":\"ConnectorPlacement.EquallySpacedRectSide\",\"uuid\":\"7ee54d08-aa3e-4d6f-8253-6f749626479a\"},{\"content\":{\"side\":\"TOP\"},\"type\":\"ConnectorPlacement.EquallySpacedRectSide\",\"uuid\":\"7bf47310-47f4-4483-b0d1-b8a087b66b77\"}]},\"type\":\"ConnectorPlacement.EquallySpacedConnector\",\"uuid\":\"fb61df21-9632-41f0-9cfa-ce5060944b6c\"}],\"packageUris\":[\"http://schema.mathworks.com/mf0/Connector/R2020b\"],\"version\":\"1.0\"}"
  CameraScheduler6 : Stateflow chart  TreatAsAtomicUnit=on
      settings: PortSchema="{\"entries\":[{\"content\":{\"sides\":[{\"content\":{\"connectorIds\":[\"In1\"]},\"type\":\"ConnectorPlacement.EquallySpacedRectSide\",\"uuid\":\"228150a7-62a2-46d0-a1ac-a8e868d835b5\"},{\"content\":{\"connectorIds\":[\"Out2\",\"Out3\",\"Out1\"],\"side\":\"RIGHT\"},\"type\":\"ConnectorPlacement.EquallySpacedRectSide\",\"uuid\":\"cb1c6840-c5bf-4913-92c2-1c054d368f87\"},{\"content\":{\"side\":\"TOP\"},\"type\":\"ConnectorPlacement.EquallySpacedRectSide\",\"uuid\":\"3633cd87-b3f9-48c9-80b7-73d7f17aa7ad\"}]},\"type\":\"ConnectorPlacement.EquallySpacedConnector\",\"uuid\":\"2553d532-cb7a-499b-b98c-b91f81677a07\"}],\"packageUris\":[\"http://schema.mathworks.com/mf0/Connector/R2020b\"],\"version\":\"1.0\"}"
  CameraScheduler7 : Stateflow chart  TreatAsAtomicUnit=on
      settings: PortSchema="{\"entries\":[{\"content\":{\"sides\":[{\"content\":{\"connectorIds\":[\"In1\"]},\"type\":\"ConnectorPlacement.EquallySpacedRectSide\",\"uuid\":\"335362b2-4c4f-40e6-baf0-d287f6971824\"},{\"content\":{\"connectorIds\":[\"Out2\",\"Out1\"],\"side\":\"RIGHT\"},\"type\":\"ConnectorPlacement.EquallySpacedRectSide\",\"uuid\":\"7ee54d08-aa3e-4d6f-8253-6f749626479a\"},{\"content\":{\"side\":\"TOP\"},\"type\":\"ConnectorPlacement.EquallySpacedRectSide\",\"uuid\":\"7bf47310-47f4-4483-b0d1-b8a087b66b77\"}]},\"type\":\"ConnectorPlacement.EquallySpacedConnector\",\"uuid\":\"fb61df21-9632-41f0-9cfa-ce5060944b6c\"}],\"packageUris\":[\"http://schema.mathworks.com/mf0/Connector/R2020b\"],\"version\":\"1.0\"}"
  CameraScheduler8 : Stateflow chart  TreatAsAtomicUnit=on
      settings: PortSchema="{\"entries\":[{\"content\":{\"sides\":[{\"content\":{\"connectorIds\":[\"In1\"]},\"type\":\"ConnectorPlacement.EquallySpacedRectSide\",\"uuid\":\"228150a7-62a2-46d0-a1ac-a8e868d835b5\"},{\"content\":{\"connectorIds\":[\"Out2\",\"Out1\"],\"side\":\"RIGHT\"},\"type\":\"ConnectorPlacement.EquallySpacedRectSide\",\"uuid\":\"cb1c6840-c5bf-4913-92c2-1c054d368f87\"},{\"content\":{\"side\":\"TOP\"},\"type\":\"ConnectorPlacement.EquallySpacedRectSide\",\"uuid\":\"3633cd87-b3f9-48c9-80b7-73d7f17aa7ad\"}]},\"type\":\"ConnectorPlacement.EquallySpacedConnector\",\"uuid\":\"2553d532-cb7a-499b-b98c-b91f81677a07\"}],\"packageUris\":[\"http://schema.mathworks.com/mf0/Connector/R2020b\"],\"version\":\"1.0\"}"
  CameraScheduler9 : Stateflow chart  TreatAsAtomicUnit=on
      settings: PortSchema="{\"entries\":[{\"content\":{\"sides\":[{\"content\":{\"connectorIds\":[\"In1\"]},\"type\":\"ConnectorPlacement.EquallySpacedRectSide\",\"uuid\":\"335362b2-4c4f-40e6-baf0-d287f6971824\"},{\"content\":{\"connectorIds\":[\"Out2\",\"Out1\"],\"side\":\"RIGHT\"},\"type\":\"ConnectorPlacement.EquallySpacedRectSide\",\"uuid\":\"7ee54d08-aa3e-4d6f-8253-6f749626479a\"},{\"content\":{\"side\":\"TOP\"},\"type\":\"ConnectorPlacement.EquallySpacedRectSide\",\"uuid\":\"7bf47310-47f4-4483-b0d1-b8a087b66b77\"}]},\"type\":\"ConnectorPlacement.EquallySpacedConnector\",\"uuid\":\"fb61df21-9632-41f0-9cfa-ce5060944b6c\"}],\"packageUris\":[\"http://schema.mathworks.com/mf0/Connector/R2020b\"],\"version\":\"1.0\"}"
  Edge : Stateflow chart  TreatAsAtomicUnit=on
  From Workspace : FromWorkspace  VariableName=arrive_time  OutDataTypeStr=double  SampleTime=-1  Interpolate=off  ZeroCross=off  OutputAfterFinalValue=Holding final value
  From Workspace1 : FromWorkspace  VariableName=visibility_time  OutDataTypeStr=double  SampleTime=-1  Interpolate=off  ZeroCross=off  OutputAfterFinalValue=Holding final value
  From Workspace10 : FromWorkspace  VariableName=timer_array_3
  From Workspace11 : FromWorkspace  VariableName=blurryness_array_4
  From Workspace12 : FromWorkspace  VariableName=networkloss_array_4
  From Workspace13 : FromWorkspace  VariableName=timer_array_4
  From Workspace14 : FromWorkspace  VariableName=timer_array_7
  From Workspace15 : FromWorkspace  VariableName=blurryness_array_8
  From Workspace16 : FromWorkspace  VariableName=networkloss_array_8
  From Workspace17 : FromWorkspace  VariableName=timer_array_8
  From Workspace18 : FromWorkspace  VariableName=blurryness_array_5
  From Workspace19 : FromWorkspace  VariableName=networkloss_array_5
  From Workspace2 : FromWorkspace  VariableName=blurryness_array_1
  From Workspace20 : FromWorkspace  VariableName=timer_array_5
  From Workspace21 : FromWorkspace  VariableName=blurryness_array_6
  From Workspace22 : FromWorkspace  VariableName=networkloss_array_6
  From Workspace23 : FromWorkspace  VariableName=timer_array_6
  From Workspace24 : FromWorkspace  VariableName=blurryness_array_7
  From Workspace25 : FromWorkspace  VariableName=networkloss_array_7
  From Workspace26 : FromWorkspace  VariableName=timer_array_11
  From Workspace27 : FromWorkspace  VariableName=blurryness_array_12
  From Workspace28 : FromWorkspace  VariableName=networkloss_array_12
  From Workspace29 : FromWorkspace  VariableName=timer_array_12
  From Workspace3 : FromWorkspace  VariableName=networkloss_array_1
  From Workspace30 : FromWorkspace  VariableName=timer_array_15
  From Workspace31 : FromWorkspace  VariableName=blurryness_array_16
  From Workspace32 : FromWorkspace  VariableName=networkloss_array_16
  From Workspace33 : FromWorkspace  VariableName=timer_array_16
  From Workspace34 : FromWorkspace  VariableName=blurryness_array_13
  From Workspace35 : FromWorkspace  VariableName=networkloss_array_13
  From Workspace36 : FromWorkspace  VariableName=blurryness_array_9
  From Workspace37 : FromWorkspace  VariableName=timer_array_13
  From Workspace38 : FromWorkspace  VariableName=blurryness_array_14
  From Workspace39 : FromWorkspace  VariableName=networkloss_array_14
  From Workspace4 : FromWorkspace  VariableName=timer_array_1
  From Workspace40 : FromWorkspace  VariableName=timer_array_14
  From Workspace41 : FromWorkspace  VariableName=blurryness_array_15
  From Workspace42 : FromWorkspace  VariableName=networkloss_array_15
  From Workspace43 : FromWorkspace  VariableName=networkloss_array_9
  From Workspace44 : FromWorkspace  VariableName=timer_array_9
  From Workspace45 : FromWorkspace  VariableName=blurryness_array_10
  From Workspace46 : FromWorkspace  VariableName=networkloss_array_10
  From Workspace47 : FromWorkspace  VariableName=timer_array_10
  From Workspace48 : FromWorkspace  VariableName=blurryness_array_11
  From Workspace49 : FromWorkspace  VariableName=networkloss_array_11
  From Workspace5 : FromWorkspace  VariableName=blurryness_array_2
  From Workspace50 : FromWorkspace  VariableName=timer_array_19
  From Workspace51 : FromWorkspace  VariableName=blurryness_array_20
  From Workspace52 : FromWorkspace  VariableName=networkloss_array_20
  From Workspace53 : FromWorkspace  VariableName=timer_array_20
  From Workspace54 : FromWorkspace  VariableName=timer_array_23
  From Workspace55 : FromWorkspace  VariableName=blurryness_array_24
  From Workspace56 : FromWorkspace  VariableName=networkloss_array_24
  From Workspace57 : FromWorkspace  VariableName=timer_array_24
  From Workspace58 : FromWorkspace  VariableName=blurryness_array_21
  From Workspace59 : FromWorkspace  VariableName=networkloss_array_21
  From Workspace6 : FromWorkspace  VariableName=networkloss_array_2
  From Workspace60 : FromWorkspace  VariableName=blurryness_array_17
  From Workspace61 : FromWorkspace  VariableName=timer_array_21
  From Workspace62 : FromWorkspace  VariableName=blurryness_array_22
  From Workspace63 : FromWorkspace  VariableName=networkloss_array_22
  From Workspace64 : FromWorkspace  VariableName=timer_array_22
  From Workspace65 : FromWorkspace  VariableName=blurryness_array_23
  From Workspace66 : FromWorkspace  VariableName=networkloss_array_23
  From Workspace67 : FromWorkspace  VariableName=timer_array_27
  From Workspace68 : FromWorkspace  VariableName=blurryness_array_28
  From Workspace69 : FromWorkspace  VariableName=networkloss_array_28
  From Workspace7 : FromWorkspace  VariableName=timer_array_2
  From Workspace70 : FromWorkspace  VariableName=timer_array_28
  From Workspace71 : FromWorkspace  VariableName=networkloss_array_17
  From Workspace72 : FromWorkspace  VariableName=timer_array_31
  From Workspace73 : FromWorkspace  VariableName=blurryness_array_32
  From Workspace74 : FromWorkspace  VariableName=networkloss_array_32
  From Workspace75 : FromWorkspace  VariableName=timer_array_32
  From Workspace76 : FromWorkspace  VariableName=blurryness_array_29
  From Workspace77 : FromWorkspace  VariableName=networkloss_array_29
  From Workspace78 : FromWorkspace  VariableName=blurryness_array_25
  From Workspace79 : FromWorkspace  VariableName=timer_array_29
  From Workspace8 : FromWorkspace  VariableName=blurryness_array_3
  From Workspace80 : FromWorkspace  VariableName=blurryness_array_30
  From Workspace81 : FromWorkspace  VariableName=networkloss_array_30
  From Workspace82 : FromWorkspace  VariableName=timer_array_17
  From Workspace83 : FromWorkspace  VariableName=timer_array_30
  From Workspace84 : FromWorkspace  VariableName=blurryness_array_31
  From Workspace85 : FromWorkspace  VariableName=networkloss_array_31
  From Workspace86 : FromWorkspace  VariableName=networkloss_array_25
  From Workspace87 : FromWorkspace  VariableName=timer_array_25
  From Workspace88 : FromWorkspace  VariableName=blurryness_array_26
  From Workspace89 : FromWorkspace  VariableName=networkloss_array_26
  From Workspace9 : FromWorkspace  VariableName=networkloss_array_3
  From Workspace90 : FromWorkspace  VariableName=timer_array_26
  From Workspace91 : FromWorkspace  VariableName=blurryness_array_27
  From Workspace92 : FromWorkspace  VariableName=networkloss_array_27
  From Workspace93 : FromWorkspace  VariableName=blurryness_array_18
  From Workspace94 : FromWorkspace  VariableName=networkloss_array_18
  From Workspace95 : FromWorkspace  VariableName=timer_array_18
  From Workspace96 : FromWorkspace  VariableName=blurryness_array_19
  From Workspace97 : FromWorkspace  VariableName=networkloss_array_19
  Scope{,1..10} (11 alike) : Scope
  To Workspace : ToWorkspace  VariableName=faults  SaveFormat=Timeseries  SampleTime=-1
  Traffic : Stateflow chart  TreatAsAtomicUnit=on
  wires:
  From Workspace/1 -> Traffic/1(arrive_time)
  From Workspace1/1 -> Traffic/2(visibility_time)
  From Workspace2/1 -> CameraDriver/3(blurryness)
  CameraControl/1(image_request) -> CameraDriver/1(image_request)
  From Workspace3/1 -> CameraControl/2(network_faults)
  From Workspace4/1 -> CameraScheduler/1(timer_array)
  CameraDriver/1(image) -> CameraControl/1(imageIn)
  Edge/1(faults) -> Scope/1, To Workspace/1
  CameraControl1/2(imageOut) -> Edge/3(image2)
  CameraDriver1/1(image) -> CameraControl1/1(imageIn)
  From Workspace7/1 -> CameraScheduler1/1(timer_array)
  From Workspace6/1 -> CameraControl1/2(network_faults)
  CameraControl1/1(image_request) -> CameraDriver1/1(image_request)
  From Workspace5/1 -> CameraDriver1/3(blurryness)
  CameraControl/2(imageOut) -> Edge/2(image1)
  CameraScheduler/1(schedule_driver) -> CameraDriver/4(schedule)
  CameraScheduler1/2(schedule_control) -> CameraControl1/3(schedule)
  CameraScheduler1/1(schedule_driver) -> CameraDriver1/4(schedule)
  CameraScheduler/2(schedule_control) -> CameraControl/3(schedule)
  Edge/2(wait_time) -> Scope1/1
  CameraScheduler/3(i) -> Scope3/1
  CameraScheduler2/3(i) -> Scope4/1
  CameraScheduler2/2(schedule_control) -> CameraControl2/3(schedule)
  CameraScheduler3/1(schedule_driver) -> CameraDriver3/4(schedule)
  CameraScheduler3/2(schedule_control) -> CameraControl3/3(schedule)
  CameraScheduler2/1(schedule_driver) -> CameraDriver2/4(schedule)
  From Workspace11/1 -> CameraDriver3/3(blurryness)
  CameraControl3/1(image_request) -> CameraDriver3/1(image_request)
  From Workspace12/1 -> CameraControl3/2(network_faults)
  From Workspace13/1 -> CameraScheduler3/1(timer_array)
  CameraDriver3/1(image) -> CameraControl3/1(imageIn)
  CameraControl3/2(imageOut) -> Edge/5(image4)
  CameraDriver2/1(image) -> CameraControl2/1(imageIn)
  From Workspace10/1 -> CameraScheduler2/1(timer_array)
  From Workspace9/1 -> CameraControl2/2(network_faults)
  CameraControl2/1(image_request) -> CameraDriver2/1(image_request)
  From Workspace8/1 -> CameraDriver2/3(blurryness)
  CameraControl2/2(imageOut) -> Edge/4(image3)
  From Workspace24/1 -> CameraDriver6/3(blurryness)
  CameraControl6/1(image_request) -> CameraDriver6/1(image_request)
  From Workspace25/1 -> CameraControl6/2(network_faults)
  From Workspace14/1 -> CameraScheduler6/1(timer_array)
  CameraDriver6/1(image) -> CameraControl6/1(imageIn)
  CameraDriver7/1(image) -> CameraControl7/1(imageIn)
  From Workspace17/1 -> CameraScheduler7/1(timer_array)
  From Workspace16/1 -> CameraControl7/2(network_faults)
  CameraControl7/1(image_request) -> CameraDriver7/1(image_request)
  From Workspace15/1 -> CameraDriver7/3(blurryness)
  CameraScheduler6/1(schedule_driver) -> CameraDriver6/4(schedule)
  CameraScheduler7/2(schedule_control) -> CameraControl7/3(schedule)
  CameraScheduler7/1(schedule_driver) -> CameraDriver7/4(schedule)
  CameraScheduler6/2(schedule_control) -> CameraControl6/3(schedule)
  CameraScheduler6/3(i) -> Scope6/1
  CameraScheduler4/3(i) -> Scope5/1
  CameraScheduler4/2(schedule_control) -> CameraControl4/3(schedule)
  CameraScheduler5/1(schedule_driver) -> CameraDriver5/4(schedule)
  CameraScheduler5/2(schedule_control) -> CameraControl5/3(schedule)
  CameraScheduler4/1(schedule_driver) -> CameraDriver4/4(schedule)
  From Workspace21/1 -> CameraDriver5/3(blurryness)
  CameraControl5/1(image_request) -> CameraDriver5/1(image_request)
  From Workspace22/1 -> CameraControl5/2(network_faults)
  From Workspace23/1 -> CameraScheduler5/1(timer_array)
  CameraDriver5/1(image) -> CameraControl5/1(imageIn)
  CameraDriver4/1(image) -> CameraControl4/1(imageIn)
  From Workspace20/1 -> CameraScheduler4/1(timer_array)
  From Workspace19/1 -> CameraControl4/2(network_faults)
  CameraControl4/1(image_request) -> CameraDriver4/1(image_request)
  From Workspace18/1 -> CameraDriver4/3(blurryness)
  CameraControl4/2(imageOut) -> Edge/6(image5)
  CameraControl5/2(imageOut) -> Edge/7(image6)
  CameraControl6/2(imageOut) -> Edge/8(image7)
  CameraControl7/2(imageOut) -> Edge/9(image8)
  From Workspace34/1 -> CameraDriver12/3(blurryness)
  CameraControl12/1(image_request) -> CameraDriver12/1(image_request)
  From Workspace35/1 -> CameraControl12/2(network_faults)
  From Workspace37/1 -> CameraScheduler12/1(timer_array)
  CameraDriver12/1(image) -> CameraControl12/1(imageIn)
  CameraDriver13/1(image) -> CameraControl13/1(imageIn)
  From Workspace40/1 -> CameraScheduler13/1(timer_array)
  From Workspace39/1 -> CameraControl13/2(network_faults)
  CameraControl13/1(image_request) -> CameraDriver13/1(image_request)
  From Workspace38/1 -> CameraDriver13/3(blurryness)
  CameraScheduler12/1(schedule_driver) -> CameraDriver12/4(schedule)
  CameraScheduler13/2(schedule_control) -> CameraControl13/3(schedule)
  CameraScheduler13/1(schedule_driver) -> CameraDriver13/4(schedule)
  CameraScheduler12/2(schedule_control) -> CameraControl12/3(schedule)
  CameraScheduler14/2(schedule_control) -> CameraControl14/3(schedule)
  CameraScheduler15/1(schedule_driver) -> CameraDriver15/4(schedule)
  CameraScheduler15/2(schedule_control) -> CameraControl15/3(schedule)
  CameraScheduler14/1(schedule_driver) -> CameraDriver14/4(schedule)
  From Workspace31/1 -> CameraDriver15/3(blurryness)
  CameraControl15/1(image_request) -> CameraDriver15/1(image_request)
  From Workspace32/1 -> CameraControl15/2(network_faults)
  From Workspace33/1 -> CameraScheduler15/1(timer_array)
  CameraDriver15/1(image) -> CameraControl15/1(imageIn)
  CameraDriver14/1(image) -> CameraControl14/1(imageIn)
  From Workspace30/1 -> CameraScheduler14/1(timer_array)
  From Workspace42/1 -> CameraControl14/2(network_faults)
  CameraControl14/1(image_request) -> CameraDriver14/1(image_request)
  From Workspace41/1 -> CameraDriver14/3(blurryness)
  From Workspace48/1 -> CameraDriver10/3(blurryness)
  CameraControl10/1(image_request) -> CameraDriver10/1(image_request)
  From Workspace49/1 -> CameraControl10/2(network_faults)
  From Workspace26/1 -> CameraScheduler10/1(timer_array)
  CameraDriver10/1(image) -> CameraControl10/1(imageIn)
  CameraDriver11/1(image) -> CameraControl11/1(imageIn)
  From Workspace29/1 -> CameraScheduler11/1(timer_array)
  From Workspace28/1 -> CameraControl11/2(network_faults)
  CameraControl11/1(image_request) -> CameraDriver11/1(image_request)
  From Workspace27/1 -> CameraDriver11/3(blurryness)
  CameraScheduler10/1(schedule_driver) -> CameraDriver10/4(schedule)
  CameraScheduler11/2(schedule_control) -> CameraControl11/3(schedule)
  CameraScheduler11/1(schedule_driver) -> CameraDriver11/4(schedule)
  CameraScheduler10/2(schedule_control) -> CameraControl10/3(schedule)
  CameraScheduler8/2(schedule_control) -> CameraControl8/3(schedule)
  CameraScheduler9/1(schedule_driver) -> CameraDriver9/4(schedule)
  CameraScheduler9/2(schedule_control) -> CameraControl9/3(schedule)
  CameraScheduler8/1(schedule_driver) -> CameraDriver8/4(schedule)
  From Workspace45/1 -> CameraDriver9/3(blurryness)
  CameraControl9/1(image_request) -> CameraDriver9/1(image_request)
  From Workspace46/1 -> CameraControl9/2(network_faults)
  From Workspace47/1 -> CameraScheduler9/1(timer_array)
  CameraDriver9/1(image) -> CameraControl9/1(imageIn)
  CameraDriver8/1(image) -> CameraControl8/1(imageIn)
  From Workspace44/1 -> CameraScheduler8/1(timer_array)
  From Workspace43/1 -> CameraControl8/2(network_faults)
  CameraControl8/1(image_request) -> CameraDriver8/1(image_request)
  From Workspace36/1 -> CameraDriver8/3(blurryness)
  CameraControl8/2(imageOut) -> Edge/10(image9)
  CameraControl9/2(imageOut) -> Edge/11(image10)
  CameraControl10/2(imageOut) -> Edge/12(image11)
  CameraControl11/2(imageOut) -> Edge/13(image12)
  CameraControl12/2(imageOut) -> Edge/14(image13)
  CameraControl13/2(imageOut) -> Edge/15(image14)
  CameraControl14/2(imageOut) -> Edge/16(image15)
  CameraControl15/2(imageOut) -> Edge/17(image16)
  From Workspace78/1 -> CameraDriver30/3(blurryness)
  CameraControl30/1(image_request) -> CameraDriver30/1(image_request)
  From Workspace86/1 -> CameraControl30/2(network_faults)
  From Workspace87/1 -> CameraScheduler30/1(timer_array)
  CameraDriver30/1(image) -> CameraControl30/1(imageIn)
  CameraDriver31/1(image) -> CameraControl31/1(imageIn)
  From Workspace90/1 -> CameraScheduler31/1(timer_array)
  From Workspace89/1 -> CameraControl31/2(network_faults)
  CameraControl31/1(image_request) -> CameraDriver31/1(image_request)
  From Workspace88/1 -> CameraDriver31/3(blurryness)
  CameraScheduler30/1(schedule_driver) -> CameraDriver30/4(schedule)
  CameraScheduler31/2(schedule_control) -> CameraControl31/3(schedule)
  CameraScheduler31/1(schedule_driver) -> CameraDriver31/4(schedule)
  CameraScheduler30/2(schedule_control) -> CameraControl30/3(schedule)
  CameraScheduler18/2(schedule_control) -> CameraControl18/3(schedule)
  CameraScheduler19/1(schedule_driver) -> CameraDriver19/4(schedule)
  CameraScheduler19/2(schedule_control) -> CameraControl19/3(schedule)
  CameraScheduler18/1(schedule_driver) -> CameraDriver18/4(schedule)
  From Workspace68/1 -> CameraDriver19/3(blurryness)
  CameraControl19/1(image_request) -> CameraDriver19/1(image_request)
  From Workspace69/1 -> CameraControl19/2(network_faults)
  From Workspace70/1 -> CameraScheduler19/1(timer_array)
  CameraDriver19/1(image) -> CameraControl19/1(imageIn)
  CameraDriver18/1(image) -> CameraControl18/1(imageIn)
  From Workspace67/1 -> CameraScheduler18/1(timer_array)
  From Workspace92/1 -> CameraControl18/2(network_faults)
  CameraControl18/1(image_request) -> CameraDriver18/1(image_request)
  From Workspace91/1 -> CameraDriver18/3(blurryness)
  From Workspace84/1 -> CameraDriver22/3(blurryness)
  CameraControl22/1(image_request) -> CameraDriver22/1(image_request)
  From Workspace85/1 -> CameraControl22/2(network_faults)
  From Workspace72/1 -> CameraScheduler22/1(timer_array)
  CameraDriver22/1(image) -> CameraControl22/1(imageIn)
  CameraDriver23/1(image) -> CameraControl23/1(imageIn)
  From Workspace75/1 -> CameraScheduler23/1(timer_array)
  From Workspace74/1 -> CameraControl23/2(network_faults)
  CameraControl23/1(image_request) -> CameraDriver23/1(image_request)
  Traffic/1(traffic_state) -> CameraDriver/2(traffic_state), CameraDriver2/2(traffic_state), CameraDriver3/2(traffic_state), CameraDriver7/2(traffic_state), CameraDriver9/2(traffic_state), CameraDriver13/2(traffic_state), CameraDriver14/2(traffic_state), CameraDriver31/2(traffic_state), CameraDriver23/2(traffic_state), CameraDriver22/2(traffic_state), CameraDriver21/2(traffic_state), CameraDriver20/2(traffic_state), CameraDriver19/2(traffic_state), CameraDriver18/2(traffic_state), CameraDriver30/2(traffic_state), CameraDriver29/2(traffic_state), CameraDriver28/2(traffic_state), CameraDriver27/2(traffic_state), CameraDriver26/2(traffic_state), CameraDriver25/2(traffic_state), CameraDriver24/2(traffic_state), CameraDriver17/2(traffic_state), CameraDriver16/2(traffic_state), CameraDriver15/2(traffic_state), CameraDriver12/2(traffic_state), CameraDriver11/2(traffic_state), CameraDriver10/2(traffic_state), CameraDriver8/2(traffic_state), CameraDriver6/2(traffic_state), CameraDriver5/2(traffic_state), CameraDriver4/2(traffic_state), CameraDriver1/2(traffic_state), Scope2/1, Edge/1(traffic_state)
  From Workspace73/1 -> CameraDriver23/3(blurryness)
  CameraScheduler22/1(schedule_driver) -> CameraDriver22/4(schedule)
  CameraScheduler23/2(schedule_control) -> CameraControl23/3(schedule)
  CameraScheduler23/1(schedule_driver) -> CameraDriver23/4(schedule)
  CameraScheduler22/2(schedule_control) -> CameraControl22/3(schedule)
  CameraScheduler20/2(schedule_control) -> CameraControl20/3(schedule)
  CameraScheduler21/1(schedule_driver) -> CameraDriver21/4(schedule)
  CameraScheduler21/2(schedule_control) -> CameraControl21/3(schedule)
  CameraScheduler20/1(schedule_driver) -> CameraDriver20/4(schedule)
  From Workspace80/1 -> CameraDriver21/3(blurryness)
  CameraControl21/1(image_request) -> CameraDriver21/1(image_request)
  From Workspace81/1 -> CameraControl21/2(network_faults)
  From Workspace83/1 -> CameraScheduler21/1(timer_array)
  CameraDriver21/1(image) -> CameraControl21/1(imageIn)
  CameraDriver20/1(image) -> CameraControl20/1(imageIn)
  From Workspace79/1 -> CameraScheduler20/1(timer_array)
  From Workspace77/1 -> CameraControl20/2(network_faults)
  CameraControl20/1(image_request) -> CameraDriver20/1(image_request)
  From Workspace76/1 -> CameraDriver20/3(blurryness)
  From Workspace58/1 -> CameraDriver26/3(blurryness)
  CameraControl26/1(image_request) -> CameraDriver26/1(image_request)
  From Workspace59/1 -> CameraControl26/2(network_faults)
  From Workspace61/1 -> CameraScheduler26/1(timer_array)
  CameraDriver26/1(image) -> CameraControl26/1(imageIn)
  CameraDriver27/1(image) -> CameraControl27/1(imageIn)
  From Workspace64/1 -> CameraScheduler27/1(timer_array)
  From Workspace63/1 -> CameraControl27/2(network_faults)
  CameraControl27/1(image_request) -> CameraDriver27/1(image_request)
  From Workspace62/1 -> CameraDriver27/3(blurryness)
  CameraScheduler26/1(schedule_driver) -> CameraDriver26/4(schedule)
  CameraScheduler27/2(schedule_control) -> CameraControl27/3(schedule)
  CameraScheduler27/1(schedule_driver) -> CameraDriver27/4(schedule)
  CameraScheduler26/2(schedule_control) -> CameraControl26/3(schedule)
  CameraScheduler26/3(i) -> Scope9/1
  CameraScheduler28/3(i) -> Scope10/1
  CameraScheduler28/2(schedule_control) -> CameraControl28/3(schedule)
  CameraScheduler29/1(schedule_driver) -> CameraDriver29/4(schedule)
  CameraScheduler29/2(schedule_control) -> CameraControl29/3(schedule)
  CameraScheduler28/1(schedule_driver) -> CameraDriver28/4(schedule)
  From Workspace55/1 -> CameraDriver29/3(blurryness)
  CameraControl29/1(image_request) -> CameraDriver29/1(image_request)
  From Workspace56/1 -> CameraControl29/2(network_faults)
  From Workspace57/1 -> CameraScheduler29/1(timer_array)
  CameraDriver29/1(image) -> CameraControl29/1(imageIn)
  CameraDriver28/1(image) -> CameraControl28/1(imageIn)
  From Workspace54/1 -> CameraScheduler28/1(timer_array)
  From Workspace66/1 -> CameraControl28/2(network_faults)
  CameraControl28/1(image_request) -> CameraDriver28/1(image_request)
  From Workspace65/1 -> CameraDriver28/3(blurryness)
  From Workspace96/1 -> CameraDriver24/3(blurryness)
  CameraControl24/1(image_request) -> CameraDriver24/1(image_request)
  From Workspace97/1 -> CameraControl24/2(network_faults)
  From Workspace50/1 -> CameraScheduler24/1(timer_array)
  CameraDriver24/1(image) -> CameraControl24/1(imageIn)
  CameraDriver25/1(image) -> CameraControl25/1(imageIn)
  From Workspace53/1 -> CameraScheduler25/1(timer_array)
  From Workspace52/1 -> CameraControl25/2(network_faults)
  CameraControl25/1(image_request) -> CameraDriver25/1(image_request)
  From Workspace51/1 -> CameraDriver25/3(blurryness)
  CameraScheduler24/1(schedule_driver) -> CameraDriver24/4(schedule)
  CameraScheduler25/2(schedule_control) -> CameraControl25/3(schedule)
  CameraScheduler25/1(schedule_driver) -> CameraDriver25/4(schedule)
  CameraScheduler24/2(schedule_control) -> CameraControl24/3(schedule)
  CameraScheduler24/3(i) -> Scope8/1
  CameraScheduler16/3(i) -> Scope7/1
  CameraScheduler16/2(schedule_control) -> CameraControl16/3(schedule)
  CameraScheduler17/1(schedule_driver) -> CameraDriver17/4(schedule)
  CameraScheduler17/2(schedule_control) -> CameraControl17/3(schedule)
  CameraScheduler16/1(schedule_driver) -> CameraDriver16/4(schedule)
  From Workspace93/1 -> CameraDriver17/3(blurryness)
  CameraControl17/1(image_request) -> CameraDriver17/1(image_request)
  From Workspace94/1 -> CameraControl17/2(network_faults)
  From Workspace95/1 -> CameraScheduler17/1(timer_array)
  CameraDriver17/1(image) -> CameraControl17/1(imageIn)
  CameraDriver16/1(image) -> CameraControl16/1(imageIn)
  From Workspace82/1 -> CameraScheduler16/1(timer_array)
  From Workspace71/1 -> CameraControl16/2(network_faults)
  CameraControl16/1(image_request) -> CameraDriver16/1(image_request)
  From Workspace60/1 -> CameraDriver16/3(blurryness)
  CameraControl16/2(imageOut) -> Edge/18(image17)
  CameraControl17/2(imageOut) -> Edge/19(image18)
  CameraControl24/2(imageOut) -> Edge/20(image19)
  CameraControl25/2(imageOut) -> Edge/21(image20)
  CameraControl26/2(imageOut) -> Edge/22(image21)
  CameraControl27/2(imageOut) -> Edge/23(image22)
  CameraControl28/2(imageOut) -> Edge/24(image23)
  CameraControl29/2(imageOut) -> Edge/25(image24)
  CameraControl30/2(imageOut) -> Edge/26(image25)
  CameraControl31/2(imageOut) -> Edge/27(image26)
  CameraControl18/2(imageOut) -> Edge/28(image27)
  CameraControl19/2(imageOut) -> Edge/29(image28)
  CameraControl20/2(imageOut) -> Edge/30(image29)
  CameraControl21/2(imageOut) -> Edge/31(image30)
  CameraControl22/2(imageOut) -> Edge/32(image31)
  CameraControl23/2(imageOut) -> Edge/33(image32)
